simulink library "ammclib_bam_S32K14x"  (R2016a)
settings: Solver=VariableStepAuto  SolverMode=SingleTasking  StartTime=0.0  StopTime=10.0  RelTol=1e-3
undefined symbols (not defined in the file or in its folder): f16A1, f16A2, f16ADCMaxError, f16B0, f16B1, f16B2, f16C1, f16CC1, f16CC1sc, f16CC1sc_D, f16CC1sc_Q, f16CC2, f16CC2sc, f16CC2sc_D, f16CC2sc_Q, f16DerivGain, f16EGain, f16FiltCoef, f16HystOff, f16HystOn, f16IGain, f16IntegGain, f16IntegGainFW, f16IntegGainQ, f16Kd, f16Kq, f16Limit, f16LowerLimit, f16LowerLimit_D, f16LowerLimit_Q, f16LowerLimitFW, f16LowerLimitQ, f16ModIndex, f16OutValOff, f16OutValOn, f16PropGain, f16PropGainFW, f16PropGainQ, f16RampDown, f16RampUp, f16UGain, f16UpperLimit, f16UpperLimit_D, f16UpperLimit_Q, f16UpperLimitFW, f16UpperLimitQ, f16WIGain, f32A1, f32A2, f32ADCMaxError, f32B0, f32B1, f32B2, f32C1, f32CC1, f32CC1sc, f32CC1sc_D, f32CC1sc_Q, f32CC2, f32CC2sc ... (+114)
(part 13 of 22)

== system ammclib_bam_S32K14x/GFLIB/FLT ==
  GFLIB_Acos_FLT : Subsystem  TreatAsAtomicUnit=on  mask(GFLIB_Acos_FLT){}
      mask help: Inverse cosine function in single precision floating-point implementation. Refer to the AMMCLIB User's Guide for further details.
      mask init: same as ammclib_bam_S32K14x/GDFLIB/F16/GDFLIB_FilterFIR_F16
      settings: RTWSystemCode=Inline
      mask Help: web([fileparts(which('ammclib_bam_S32K14x.slx')) '/../doc/S32K14XMCLUG.pdf'], '-browser')
      mask Display: pos = get_param(gcb, 'Position');width = pos(3) - pos(1); height = pos(4) - pos(2);tX=width/2;tY=height - 8;color('black');text(tX,tY, 'GFLIB_Acos_FLT', 'horizontalAlignment', 'center');
  GFLIB_Asin_FLT : Subsystem  TreatAsAtomicUnit=on  mask(GFLIB_Asin_FLT){}
      mask help: Inverse sine function in single precision floating-point implementation. Refer to the AMMCLIB User's Guide for further details.
      mask init: same as ammclib_bam_S32K14x/GDFLIB/F16/GDFLIB_FilterFIR_F16
      settings: RTWSystemCode=Inline
      mask Help: web([fileparts(which('ammclib_bam_S32K14x.slx')) '/../doc/S32K14XMCLUG.pdf'], '-browser')
      mask Display: pos = get_param(gcb, 'Position');width = pos(3) - pos(1); height = pos(4) - pos(2);tX=width/2;tY=height - 8;color('black');text(tX,tY, 'GFLIB_Asin_FLT', 'horizontalAlignment', 'center');
  GFLIB_AtanYXShifted_FLT : Subsystem  TreatAsAtomicUnit=on  mask(GFLIB_AtanYXShifted_FLT){}
      mask help: Shifted arctangent of two arguments Y/X in single precision floating-point implementation. Refer to the AMMCLIB User's Guide for further details.
      mask init: same as ammclib_bam_S32K14x/GDFLIB/F16/GDFLIB_FilterFIR_F16
      settings: RTWSystemCode=Inline
      mask Help: web([fileparts(which('ammclib_bam_S32K14x.slx')) '/../doc/S32K14XMCLUG.pdf'], '-browser')
      mask Display: pos = get_param(gcb, 'Position');width = pos(3) - pos(1); height = pos(4) - pos(2);tX=width/2;tY=height - 8;color('black');text(tX,tY, 'GFLIB_AtanYXShifted_FLT', 'horizontalAlignment', 'center');
  GFLIB_AtanYX_FLT : Subsystem  TreatAsAtomicUnit=on  mask(GFLIB_AtanYX_FLT){}
      mask help: Arctangent of two arguments Y/X in single precision floating-point implementation. Refer to the AMMCLIB User's Guide for further details.
      mask init: same as ammclib_bam_S32K14x/GDFLIB/F16/GDFLIB_FilterFIR_F16
      settings: RTWSystemCode=Inline
      mask Help: web([fileparts(which('ammclib_bam_S32K14x.slx')) '/../doc/S32K14XMCLUG.pdf'], '-browser')
      mask Display: pos = get_param(gcb, 'Position');width = pos(3) - pos(1); height = pos(4) - pos(2);tX=width/2;tY=height - 8;color('black');text(tX,tY, 'GFLIB_AtanYX_FLT', 'horizontalAlignment', 'center');
  GFLIB_Atan_FLT : Subsystem  TreatAsAtomicUnit=on  mask(GFLIB_Atan_FLT){}
      mask help: Inverse tangent function in single precision floating-point implementation. Refer to the AMMCLIB User's Guide for further details.
      mask init: same as ammclib_bam_S32K14x/GDFLIB/F16/GDFLIB_FilterFIR_F16
      settings: RTWSystemCode=Inline
      mask Help: web([fileparts(which('ammclib_bam_S32K14x.slx')) '/../doc/S32K14XMCLUG.pdf'], '-browser')
      mask Display: pos = get_param(gcb, 'Position');width = pos(3) - pos(1); height = pos(4) - pos(2);tX=width/2;tY=height - 8;color('black');text(tX,tY, 'GFLIB_Atan_FLT', 'horizontalAlignment', 'center');
  GFLIB_ControllerPIDpAW_FLT : Subsystem  TreatAsAtomicUnit=on  mask(GFLIB_ControllerPIDpAW_FLT){showStates=Hide (faster execution), resetStatesEnable=Pre-set according to the first set of inputs after reset, fltPropGain=0, fltIntegGain=0, fltDerivGain=0, fltFiltCoef=0, fltLowerLimit=0, fltUpperLimit=0}
      mask prompts: showStates "Show internal states"; resetStatesEnable "Internal state after reset"; fltPropGain "fltPropGain (Proportional gain)"; fltIntegGain "fltIntegGain (Integral gain)"; fltDerivGain "fltDerivGain (Derivative Gain)"; fltFiltCoef "fltFiltCoef (Derivative term filter coefficient)"; fltLowerLimit "fltLowerLimit (Lower Limit of the controller)"; fltUpperLimit "fltUpperLimit (Upper Limit of the controller)"
      mask help: Parallel form PID controller with anti-windup in single precision floating-point implementation. This block supports re-initialization of the internal state during simulation. If the block is reset, the controller's output will be aligned with the input fltControllerPIDpAWOut_preset. Refer to the AMMCLIB User's Guide for further details.
      mask init:
      | if ~evalin('base','exist(''tS8'',''var'')')
      |   if (2 ~= exist('SWLIBS_Typedefs.mat','file'))
      |       error('File SWLIBS_Typedefs.mat is not on the Matlab path. Please add the AMMCLIB "bam" folder in the Matlab Search Path.');
      |   else
      |       evalin('base', 'load(''SWLIBS_Typedefs.mat'')');
      |   end
      | end
      | if showStates == 1
      |     % hidden state variables
      |     if strcmp(get_param([gcb '/fltPropGain'], 'BlockType'), 'Inport')
      |         posblk = get_param(gcb, 'Position');
      | 
      |         pos = get_param(    [gcb, '/fltPropGain'], 'Position');
      |         orient = get_param( [gcb, '/fltPropGain'], 'Orientation');
      |         delete_block(       [gcb, '/fltPropGain']);
      |         add_block('built-in/Ground', [gcb, '/fltPropGain'], 'Position', pos, 'Orientation', orient);
      | 
      |         pos = get_param(    [gcb, '/fltIntegGain'], 'Position');
      |         orient = get_param( [gcb, '/fltIntegGain'], 'Orientation');
      |         delete_block(       [gcb, '/fltIntegGain']);
      |         add_block('built-in/Ground', [gcb, '/fltIntegGain'], 'Position', pos, 'Orientation', orient);
      | 
      |         pos = get_param(    [gcb, '/fltDerivGain'], 'Position');
      |         orient = get_param( [gcb, '/fltDerivGain'], 'Orientation');
      |         delete_block(       [gcb, '/fltDerivGain']);
      |         add_block('built-in/Ground', [gcb, '/fltDerivGain'], 'Position', pos, 'Orientation', orient);
      | 
      |         pos = get_param(    [gcb, '/fltFiltCoef'], 'Position');
      |         orient = get_param( [gcb, '/fltFiltCoef'], 'Orientation');
      |         delete_block(       [gcb, '/fltFiltCoef']);
      |         add_block('built-in/Ground', [gcb, '/fltFiltCoef'], 'Position', pos, 'Orientation', orient);
      | 
      |         pos = get_param(    [gcb, '/fltLowerLimit'], 'Position');
      |         orient = get_param( [gcb, '/fltLowerLimit'], 'Orientation');
      |         delete_block(       [gcb, '/fltLowerLimit']);
      |         add_block('built-in/Ground', [gcb, '/fltLowerLimit'], 'Position', pos, 'Orientation', orient);
      | 
      |         pos = get_param(    [gcb, '/fltUpperLimit'], 'Position');
      |         orient = get_param( [gcb, '/fltUpperLimit'], 'Orientation');
      |         delete_block(       [gcb, '/fltUpperLimit']);
      |         add_block('built-in/Ground', [gcb, '/fltUpperLimit'], 'Position', pos, 'Orientation', orient);
      | 
      |         pos = get_param(    [gcb, '/fltIntegPartK_1'], 'Position');
      |         orient = get_param( [gcb, '/fltIntegPartK_1'], 'Orientation');
      |         delete_block(       [gcb, '/fltIntegPartK_1']);
      |         add_block('built-in/Ground', [gcb, '/fltIntegPartK_1'], 'Position', pos, 'Orientation', orient);
      | 
      |         pos = get_param(    [gcb, '/fltDerivPartK_1'], 'Position');
      |         orient = get_param( [gcb, '/fltDerivPartK_1'], 'Orientation');
      |         delete_block(       [gcb, '/fltDerivPartK_1']);
      |         add_block('built-in/Ground', [gcb, '/fltDerivPartK_1'], 'Position', pos, 'Orientation', orient);
      | 
      |         pos = get_param(    [gcb, '/fltInK_1'], 'Position');
      |         orient = get_param( [gcb, '/fltInK_1'], 'Orientation');
      |         delete_block(       [gcb, '/fltInK_1']);
      |         add_block('built-in/Ground', [gcb, '/fltInK_1'], 'Position', pos, 'Orientation', orient);
      | 
      | 
      |         pos = get_param(    [gcb '/fltIntegPartK_1_Out'], 'Position');
      |         orient = get_param( [gcb '/fltIntegPartK_1_Out'], 'Orientation');
      |         delete_block(       [gcb '/fltIntegPartK_1_Out']);
      |         add_block('built-in/Terminator', [gcb '/fltIntegPartK_1_Out'], 'Position', pos, 'Orientation', orient);
      | 
      |         pos = get_param(    [gcb '/fltDerivPartK_1_Out'], 'Position');
      |         orient = get_param( [gcb '/fltDerivPartK_1_Out'], 'Orientation');
      |         delete_block(       [gcb '/fltDerivPartK_1_Out']);
      |         add_block('built-in/Terminator', [gcb '/fltDerivPartK_1_Out'], 'Position', pos, 'Orientation', orient);
      | 
      |         pos = get_param(    [gcb '/fltInK_1_Out'], 'Position');
      |         orient = get_param( [gcb '/fltInK_1_Out'], 'Orientation');
      |         delete_block(       [gcb '/fltInK_1_Out']);
      |         add_block('built-in/Terminator', [gcb '/fltInK_1_Out'], 'Position', pos, 'Orientation', orient);
      | 
      | 
      |         set_param([gcb '/fltInErr'], 'Port', '1');
      |         set_param([gcb '/fltControllerPIDpAWOut_preset'], 'Port', '2');
      | 
      |         set_param([gcb '/fltOut'], 'Port', '1');
      |         set_param([gcb '/u16LimitFlag'], 'Port', '2');
      | 
      |         set_param(gcb,'MaskEnables',{'on','on','on','on','on','on','on','on'});
      | 
      |         if (posblk(4) - posblk(2)) > 75
      |           height = 75;
      |           set_param(gcb,'Position',[posblk(1), posblk(2), posblk(3), posblk(2)+height])
      |         end
      |     end
      | else
      |     % shown state variables
      |     if strcmp(get_param([gcb '/fltPropGain'], 'BlockType'), 'Ground')
      |         posblk = get_param(gcb, 'Position');
      | 
      |         pos = get_param(    [gcb, '/fltPropGain'], 'Position');
      |         orient = get_param( [gcb, '/fltPropGain'], 'Orientation');
      |         delete_block(       [gcb, '/fltPropGain']);
      |         add_block('built-in/Inport', [gcb, '/fltPropGain'], 'Position', pos, 'Orientation', orient, 'OutDataTypeStr', 'single');
      | 
      |         pos = get_param(    [gcb, '/fltIntegGain'], 'Position');
      |         orient = get_param( [gcb, '/fltIntegGain'], 'Orientation');
      |         delete_block(       [gcb, '/fltIntegGain']);
      |         add_block('built-in/Inport', [gcb, '/fltIntegGain'], 'Position', pos, 'Orientation', orient, 'OutDataTypeStr', 'single');
      | 
      |         pos = get_param(    [gcb, '/fltDerivGain'], 'Position');
      |         orient = get_param( [gcb, '/fltDerivGain'], 'Orientation');
      |         delete_block(       [gcb, '/fltDerivGain']);
      |         add_block('built-in/Inport', [gcb, '/fltDerivGain'], 'Position', pos, 'Orientation', orient, 'OutDataTypeStr', 'single');
      | 
      |         pos = get_param(    [gcb, '/fltFiltCoef'], 'Position');
      |         orient = get_param( [gcb, '/fltFiltCoef'], 'Orientation');
      |         delete_block(       [gcb, '/fltFiltCoef']);
      |         add_block('built-in/Inport', [gcb, '/fltFiltCoef'], 'Position', pos, 'Orientation', orient, 'OutDataTypeStr', 'single');
      | 
      |         pos = get_param(    [gcb, '/fltLowerLimit'], 'Position');
      |         orient = get_param( [gcb, '/fltLowerLimit'], 'Orientation');
      |         delete_block(       [gcb, '/fltLowerLimit']);
      |         add_block('built-in/Inport', [gcb, '/fltLowerLimit'], 'Position', pos, 'Orientation', orient, 'OutDataTypeStr', 'single');
      | 
      |         pos = get_param(    [gcb, '/fltUpperLimit'], 'Position');
      |         orient = get_param( [gcb, '/fltUpperLimit'], 'Orientation');
      |         delete_block(       [gcb, '/fltUpperLimit']);
      |         add_block('built-in/Inport', [gcb, '/fltUpperLimit'], 'Position', pos, 'Orientation', orient, 'OutDataTypeStr', 'single');
      | 
      |         pos = get_param(    [gcb, '/fltIntegPartK_1'], 'Position');
      |         orient = get_param( [gcb, '/fltIntegPartK_1'], 'Orientation');
      |         delete_block(       [gcb, '/fltIntegPartK_1']);
      |         add_block('built-in/Inport', [gcb, '/fltIntegPartK_1'], 'Position', pos, 'Orientation', orient, 'OutDataTypeStr', 'single');
      | 
      |         pos = get_param(    [gcb, '/fltDerivPartK_1'], 'Position');
      |         orient = get_param( [gcb, '/fltDerivPartK_1'], 'Orientation');
      |         delete_block(       [gcb, '/fltDerivPartK_1']);
      |         add_block('built-in/Inport', [gcb, '/fltDerivPartK_1'], 'Position', pos, 'Orientation', orient, 'OutDataTypeStr', 'single');
      | 
      |         pos = get_param(    [gcb, '/fltInK_1'], 'Position');
      |         orient = get_param( [gcb, '/fltInK_1'], 'Orientation');
      |         delete_block(       [gcb, '/fltInK_1']);
      |         add_block('built-in/Inport', [gcb, '/fltInK_1'], 'Position', pos, 'Orientation', orient, 'OutDataTypeStr', 'single');
      | 
      | 
      |         pos = get_param(    [gcb '/fltIntegPartK_1_Out'], 'Position');
      |         orient = get_param( [gcb '/fltIntegPartK_1_Out'], 'Orientation');
      |         delete_block(       [gcb '/fltIntegPartK_1_Out']);
      |         add_block('built-in/Outport', [gcb '/fltIntegPartK_1_Out'], 'Position', pos, 'Orientation', orient);
      | 
      |         pos = get_param(    [gcb '/fltDerivPartK_1_Out'], 'Position');
      |         orient = get_param( [gcb '/fltDerivPartK_1_Out'], 'Orientation');
      |         delete_block(       [gcb '/fltDerivPartK_1_Out']);
      |         add_block('built-in/Outport', [gcb '/fltDerivPartK_1_Out'], 'Position', pos, 'Orientation', orient);
      | 
      |         pos = get_param(    [gcb '/fltInK_1_Out'], 'Position');
      |         orient = get_param( [gcb '/fltInK_1_Out'], 'Orientation');
      |         delete_block(       [gcb '/fltInK_1_Out']);
      |         add_block('built-in/Outport', [gcb '/fltInK_1_Out'], 'Position', pos, 'Orientation', orient);
      | 
      | 
      |         set_param([gcb '/fltInErr'], 'Port', '1');
      |         set_param([gcb '/fltControllerPIDpAWOut_preset'], 'Port', '2');
      |         set_param([gcb '/fltPropGain'], 'Port', '3');
      |         set_param([gcb '/fltIntegGain'], 'Port', '4');
      |         set_param([gcb '/fltDerivGain'], 'Port', '5');
      |         set_param([gcb '/fltFiltCoef'], 'Port', '6');
      |         set_param([gcb '/fltLowerLimit'], 'Port', '7');
      |         set_param([gcb '/fltUpperLimit'], 'Port', '8');
      |         set_param([gcb '/fltIntegPartK_1'], 'Port', '9');
      |         set_param([gcb '/fltDerivPartK_1'], 'Port', '10');
      |         set_param([gcb '/fltInK_1'], 'Port', '11');
      | 
      |         set_param([gcb '/fltOut'], 'Port', '1');
      |         set_param([gcb '/u16LimitFlag'], 'Port', '2');
      |         set_param([gcb '/fltIntegPartK_1_Out'], 'Port', '3');
      |         set_param([gcb '/fltDerivPartK_1_Out'], 'Port', '4');
      |         set_param([gcb '/fltInK_1_Out'], 'Port', '5');
      | 
      |         set_param(gcb,'MaskEnables',{'on','on','off','off','off','off','off','off'});
      | 
      |         if (posblk(4) - posblk(2)) < 300
      |           height = 300;
      |           set_param(gcb,'Position',[posblk(1), posblk(2), posblk(3), posblk(2)+height])
      |         end
      |     end
      | end
      settings: RTWSystemCode=Inline
      mask Help: web([fileparts(which('ammclib_bam_S32K14x.slx')) '/../doc/S32K14XMCLUG.pdf'], '-browser')
      mask TypeOptions showStates: Hide (faster execution) | Show (allows debugging; connect feedback loops manually)
      mask Callback showStates:
      | maskStr = get_param(gcb,'showStates');
      | if strcmp(maskStr,'Hide (faster execution)'),
      |     set_param(gcb,'MaskEnables',{'on','on','on','on','on','on','on','on'});
      | else
      |     set_param(gcb,'MaskEnables',{'on','on','off','off','off','off','off','off'});
      | end
      mask TypeOptions resetStatesEnable: Pre-set according to the first set of inputs after reset | Clear to zero
      mask Display:
      | color('black');
      | pos = get_param(gcb, 'Position');
      | width = pos(3) - pos(1);
      | height = pos(4) - pos(2);
      | tX=width/2;
      | tY=height - 25;
      | color('black');
      | text(tX,tY, 'GFLIB_ControllerPIDpAW_FLT', 'horizontalAlignment', 'center');
      | if showStates == 2
      |   color('red');
      |   text(tX,tY - 20, ['debugging mode' char(13) char(10) '(limited performance)'], 'horizontalAlignment', 'center');
      | end
  GFLIB_ControllerPIpAW_FLT : Subsystem  TreatAsAtomicUnit=on  mask(GFLIB_ControllerPIpAW_FLT){showStates=Hide (faster execution), resetStatesEnable=Pre-set according to the first set of inputs after reset, fltPropGain=0, fltIntegGain=0, fltLowerLimit=0, fltUpperLimit=0}
      mask prompts: showStates "Show internal states"; resetStatesEnable "Internal state after reset"; fltPropGain "fltPropGain (Proportional gain)"; fltIntegGain "fltIntegGain (Integral gain)"; fltLowerLimit "fltLowerLimit (Lower Limit of the controller)"; fltUpperLimit "fltUpperLimit (Upper Limit of the controller)"
      mask help: Parallel form PI controller with anti-windup in single precision floating-point implementation. This block supports re-initialization of the internal state during simulation. If the block is reset, the controller's output will be aligned with the input fltControllerPIpAWOut_preset. Refer to the AMMCLIB User's Guide for further details.
      mask init:
      | if ~evalin('base','exist(''tS8'',''var'')')
      |   if (2 ~= exist('SWLIBS_Typedefs.mat','file'))
      |       error('File SWLIBS_Typedefs.mat is not on the Matlab path. Please add the AMMCLIB "bam" folder in the Matlab Search Path.');
      |   else
      |       evalin('base', 'load(''SWLIBS_Typedefs.mat'')');
      |   end
      | end
      | if showStates == 1
      |     % hidden state variables
      |     if strcmp(get_param([gcb '/fltPropGain'], 'BlockType'), 'Inport')
      |         posblk = get_param(gcb, 'Position');
      | 
      |         pos = get_param(    [gcb, '/fltPropGain'], 'Position');
      |         orient = get_param( [gcb, '/fltPropGain'], 'Orientation');
      |         delete_block(       [gcb, '/fltPropGain']);
      |         add_block('built-in/Ground', [gcb, '/fltPropGain'], 'Position', pos, 'Orientation', orient);
      | 
      |         pos = get_param(    [gcb, '/fltIntegGain'], 'Position');
      |         orient = get_param( [gcb, '/fltIntegGain'], 'Orientation');
      |         delete_block(       [gcb, '/fltIntegGain']);
      |         add_block('built-in/Ground', [gcb, '/fltIntegGain'], 'Position', pos, 'Orientation', orient);
      | 
      |         pos = get_param(    [gcb, '/fltLowerLimit'], 'Position');
      |         orient = get_param( [gcb, '/fltLowerLimit'], 'Orientation');
      |         delete_block(       [gcb, '/fltLowerLimit']);
      |         add_block('built-in/Ground', [gcb, '/fltLowerLimit'], 'Position', pos, 'Orientation', orient);
      | 
      |         pos = get_param(    [gcb, '/fltUpperLimit'], 'Position');
      |         orient = get_param( [gcb, '/fltUpperLimit'], 'Orientation');
      |         delete_block(       [gcb, '/fltUpperLimit']);
      |         add_block('built-in/Ground', [gcb, '/fltUpperLimit'], 'Position', pos, 'Orientation', orient);
      | 
      |         pos = get_param(    [gcb, '/fltIntegPartK_1'], 'Position');
      |         orient = get_param( [gcb, '/fltIntegPartK_1'], 'Orientation');
      |         delete_block(       [gcb, '/fltIntegPartK_1']);
      |         add_block('built-in/Ground', [gcb, '/fltIntegPartK_1'], 'Position', pos, 'Orientation', orient);
      | 
      |         pos = get_param(    [gcb, '/fltInK_1'], 'Position');
      |         orient = get_param( [gcb, '/fltInK_1'], 'Orientation');
      |         delete_block(       [gcb, '/fltInK_1']);
      |         add_block('built-in/Ground', [gcb, '/fltInK_1'], 'Position', pos, 'Orientation', orient);
      | 
      | 
      |         pos = get_param(    [gcb '/fltIntegPartK_1_Out'], 'Position');
      |         orient = get_param( [gcb '/fltIntegPartK_1_Out'], 'Orientation');
      |         delete_block(       [gcb '/fltIntegPartK_1_Out']);
      |         add_block('built-in/Terminator', [gcb '/fltIntegPartK_1_Out'], 'Position', pos, 'Orientation', orient);
      | 
      |         pos = get_param(    [gcb '/fltInK_1_Out'], 'Position');
      |         orient = get_param( [gcb '/fltInK_1_Out'], 'Orientation');
      |         delete_block(       [gcb '/fltInK_1_Out']);
      |         add_block('built-in/Terminator', [gcb '/fltInK_1_Out'], 'Position', pos, 'Orientation', orient);
      | 
      | 
      |         set_param([gcb '/fltInErr'], 'Port', '1');
      |         set_param([gcb '/fltControllerPIpAWOut_preset'], 'Port', '2');
      | 
      |         set_param([gcb '/fltOut'], 'Port', '1');
      |         set_param([gcb '/u16LimitFlag'], 'Port', '2');
      | 
      |         set_param(gcb,'MaskEnables',{'on','on','on','on','on','on'});
      | 
      |         if (posblk(4) - posblk(2)) > 75
      |           height = 75;
      |           set_param(gcb,'Position',[posblk(1), posblk(2), posblk(3), posblk(2)+height])
      |         end
      |     end
      | else
      |     % shown state variables
      |     if strcmp(get_param([gcb '/fltPropGain'], 'BlockType'), 'Ground')
      |         posblk = get_param(gcb, 'Position');
      | 
      |         pos = get_param(    [gcb, '/fltPropGain'], 'Position');
      |         orient = get_param( [gcb, '/fltPropGain'], 'Orientation');
      |         delete_block(       [gcb, '/fltPropGain']);
      |         add_block('built-in/Inport', [gcb, '/fltPropGain'], 'Position', pos, 'Orientation', orient, 'OutDataTypeStr', 'single');
      | 
      |         pos = get_param(    [gcb, '/fltIntegGain'], 'Position');
      |         orient = get_param( [gcb, '/fltIntegGain'], 'Orientation');
      |         delete_block(       [gcb, '/fltIntegGain']);
      |         add_block('built-in/Inport', [gcb, '/fltIntegGain'], 'Position', pos, 'Orientation', orient, 'OutDataTypeStr', 'single');
      | 
      |         pos = get_param(    [gcb, '/fltLowerLimit'], 'Position');
      |         orient = get_param( [gcb, '/fltLowerLimit'], 'Orientation');
      |         delete_block(       [gcb, '/fltLowerLimit']);
      |         add_block('built-in/Inport', [gcb, '/fltLowerLimit'], 'Position', pos, 'Orientation', orient, 'OutDataTypeStr', 'single');
      | 
      |         pos = get_param(    [gcb, '/fltUpperLimit'], 'Position');
      |         orient = get_param( [gcb, '/fltUpperLimit'], 'Orientation');
      |         delete_block(       [gcb, '/fltUpperLimit']);
      |         add_block('built-in/Inport', [gcb, '/fltUpperLimit'], 'Position', pos, 'Orientation', orient, 'OutDataTypeStr', 'single');
      | 
      |         pos = get_param(    [gcb, '/fltIntegPartK_1'], 'Position');
      |         orient = get_param( [gcb, '/fltIntegPartK_1'], 'Orientation');
      |         delete_block(       [gcb, '/fltIntegPartK_1']);
      |         add_block('built-in/Inport', [gcb, '/fltIntegPartK_1'], 'Position', pos, 'Orientation', orient, 'OutDataTypeStr', 'single');
      | 
      |         pos = get_param(    [gcb, '/fltInK_1'], 'Position');
      |         orient = get_param( [gcb, '/fltInK_1'], 'Orientation');
      |         delete_block(       [gcb, '/fltInK_1']);
      |         add_block('built-in/Inport', [gcb, '/fltInK_1'], 'Position', pos, 'Orientation', orient, 'OutDataTypeStr', 'single');
      | 
      | 
      |         pos = get_param(    [gcb '/fltIntegPartK_1_Out'], 'Position');
      |         orient = get_param( [gcb '/fltIntegPartK_1_Out'], 'Orientation');
      |         delete_block(       [gcb '/fltIntegPartK_1_Out']);
      |         add_block('built-in/Outport', [gcb '/fltIntegPartK_1_Out'], 'Position', pos, 'Orientation', orient);
      | 
      |         pos = get_param(    [gcb '/fltInK_1_Out'], 'Position');
      |         orient = get_param( [gcb '/fltInK_1_Out'], 'Orientation');
      |         delete_block(       [gcb '/fltInK_1_Out']);
      |         add_block('built-in/Outport', [gcb '/fltInK_1_Out'], 'Position', pos, 'Orientation', orient);
      | 
      | 
      |         set_param([gcb '/fltInErr'], 'Port', '1');
      |         set_param([gcb '/fltControllerPIpAWOut_preset'], 'Port', '2');
      |         set_param([gcb '/fltPropGain'], 'Port', '3');
      |         set_param([gcb '/fltIntegGain'], 'Port', '4');
      |         set_param([gcb '/fltLowerLimit'], 'Port', '5');
      |         set_param([gcb '/fltUpperLimit'], 'Port', '6');
      |         set_param([gcb '/fltIntegPartK_1'], 'Port', '7');
      |         set_param([gcb '/fltInK_1'], 'Port', '8');
      | 
      |         set_param([gcb '/fltOut'], 'Port', '1');
      |         set_param([gcb '/u16LimitFlag'], 'Port', '2');
      |         set_param([gcb '/fltIntegPartK_1_Out'], 'Port', '3');
      |         set_param([gcb '/fltInK_1_Out'], 'Port', '4');
      | 
      |         set_param(gcb,'MaskEnables',{'on','on','off','off','off','off'});
      | 
      |         if (posblk(4) - posblk(2)) < 225
      |           height = 225;
      |           set_param(gcb,'Position',[posblk(1), posblk(2), posblk(3), posblk(2)+height])
      |         end
      |     end
      | end
      settings: RTWSystemCode=Inline
      mask Help: web([fileparts(which('ammclib_bam_S32K14x.slx')) '/../doc/S32K14XMCLUG.pdf'], '-browser')
      mask TypeOptions showStates: Hide (faster execution) | Show (allows debugging; connect feedback loops manually)
      mask Callback showStates:
      | maskStr = get_param(gcb,'showStates');
      | if strcmp(maskStr,'Hide (faster execution)'),
      |     set_param(gcb,'MaskEnables',{'on','on','on','on','on','on'});
      | else
      |     set_param(gcb,'MaskEnables',{'on','on','off','off','off','off'});
      | end
      mask TypeOptions resetStatesEnable: Pre-set according to the first set of inputs after reset | Clear to zero
      mask Display:
      | color('black');
      | pos = get_param(gcb, 'Position');
      | width = pos(3) - pos(1);
      | height = pos(4) - pos(2);
      | tX=width/2;
      | tY=height - 25;
      | color('black');
      | text(tX,tY, 'GFLIB_ControllerPIpAW_FLT', 'horizontalAlignment', 'center');
      | if showStates == 2
      |   color('red');
      |   text(tX,tY - 20, ['debugging mode' char(13) char(10) '(limited performance)'], 'horizontalAlignment', 'center');
      | end
  GFLIB_ControllerPIp_FLT : Subsystem  TreatAsAtomicUnit=on  mask(GFLIB_ControllerPIp_FLT){showStates=Hide (faster execution), resetStatesEnable=Pre-set according to the first set of inputs after reset, fltPropGain=0, fltIntegGain=0}
      mask prompts: showStates "Show internal states"; resetStatesEnable "Internal state after reset"; fltPropGain "fltPropGain (Proportional gain)"; fltIntegGain "fltIntegGain (Integral gain)"
      mask help: Parallel form PI controller without anti-windup in single precision floating-point implementation. This block supports re-initialization of the internal state during simulation. If the block is reset, the controller's output will be aligned with the input fltControllerPIpOut_preset. Refer to the AMMCLIB User's Guide for further details.
      mask init:
      | if ~evalin('base','exist(''tS8'',''var'')')
      |   if (2 ~= exist('SWLIBS_Typedefs.mat','file'))
      |       error('File SWLIBS_Typedefs.mat is not on the Matlab path. Please add the AMMCLIB "bam" folder in the Matlab Search Path.');
      |   else
      |       evalin('base', 'load(''SWLIBS_Typedefs.mat'')');
      |   end
      | end
      | if showStates == 1
      |     % hidden state variables
      |     if strcmp(get_param([gcb '/fltPropGain'], 'BlockType'), 'Inport')
      |         posblk = get_param(gcb, 'Position');
      | 
      |         pos = get_param(    [gcb, '/fltPropGain'], 'Position');
      |         orient = get_param( [gcb, '/fltPropGain'], 'Orientation');
      |         delete_block(       [gcb, '/fltPropGain']);
      |         add_block('built-in/Ground', [gcb, '/fltPropGain'], 'Position', pos, 'Orientation', orient);
      | 
      |         pos = get_param(    [gcb, '/fltIntegGain'], 'Position');
      |         orient = get_param( [gcb, '/fltIntegGain'], 'Orientation');
      |         delete_block(       [gcb, '/fltIntegGain']);
      |         add_block('built-in/Ground', [gcb, '/fltIntegGain'], 'Position', pos, 'Orientation', orient);
      | 
      |         pos = get_param(    [gcb, '/fltIntegPartK_1'], 'Position');
      |         orient = get_param( [gcb, '/fltIntegPartK_1'], 'Orientation');
      |         delete_block(       [gcb, '/fltIntegPartK_1']);
      |         add_block('built-in/Ground', [gcb, '/fltIntegPartK_1'], 'Position', pos, 'Orientation', orient);
      | 
      |         pos = get_param(    [gcb, '/fltInK_1'], 'Position');
      |         orient = get_param( [gcb, '/fltInK_1'], 'Orientation');
      |         delete_block(       [gcb, '/fltInK_1']);
      |         add_block('built-in/Ground', [gcb, '/fltInK_1'], 'Position', pos, 'Orientation', orient);
      | 
      | 
      |         pos = get_param(    [gcb '/fltIntegPartK_1_Out'], 'Position');
      |         orient = get_param( [gcb '/fltIntegPartK_1_Out'], 'Orientation');
      |         delete_block(       [gcb '/fltIntegPartK_1_Out']);
      |         add_block('built-in/Terminator', [gcb '/fltIntegPartK_1_Out'], 'Position', pos, 'Orientation', orient);
      | 
      |         pos = get_param(    [gcb '/fltInK_1_Out'], 'Position');
      |         orient = get_param( [gcb '/fltInK_1_Out'], 'Orientation');
      |         delete_block(       [gcb '/fltInK_1_Out']);
      |         add_block('built-in/Terminator', [gcb '/fltInK_1_Out'], 'Position', pos, 'Orientation', orient);
      | 
      | 
      |         set_param([gcb '/fltInErr'], 'Port', '1');
      |         set_param([gcb '/fltControllerPIpOut_preset'], 'Port', '2');
      | 
      |         set_param([gcb '/fltOut'], 'Port', '1');
      | 
      |         set_param(gcb,'MaskEnables',{'on','on','on','on'});
      | 
      |         if (posblk(4) - posblk(2)) > 75
      |           height = 75;
      |           set_param(gcb,'Position',[posblk(1), posblk(2), posblk(3), posblk(2)+height])
      |         end
      |     end
      | else
      |     % shown state variables
      |     if strcmp(get_param([gcb '/fltPropGain'], 'BlockType'), 'Ground')
      |         posblk = get_param(gcb, 'Position');
      | 
      |         pos = get_param(    [gcb, '/fltPropGain'], 'Position');
      |         orient = get_param( [gcb, '/fltPropGain'], 'Orientation');
      |         delete_block(       [gcb, '/fltPropGain']);
      |         add_block('built-in/Inport', [gcb, '/fltPropGain'], 'Position', pos, 'Orientation', orient, 'OutDataTypeStr', 'single');
      | 
      |         pos = get_param(    [gcb, '/fltIntegGain'], 'Position');
      |         orient = get_param( [gcb, '/fltIntegGain'], 'Orientation');
      |         delete_block(       [gcb, '/fltIntegGain']);
      |         add_block('built-in/Inport', [gcb, '/fltIntegGain'], 'Position', pos, 'Orientation', orient, 'OutDataTypeStr', 'single');
      | 
      |         pos = get_param(    [gcb, '/fltIntegPartK_1'], 'Position');
      |         orient = get_param( [gcb, '/fltIntegPartK_1'], 'Orientation');
      |         delete_block(       [gcb, '/fltIntegPartK_1']);
      |         add_block('built-in/Inport', [gcb, '/fltIntegPartK_1'], 'Position', pos, 'Orientation', orient, 'OutDataTypeStr', 'single');
      | 
      |         pos = get_param(    [gcb, '/fltInK_1'], 'Position');
      |         orient = get_param( [gcb, '/fltInK_1'], 'Orientation');
      |         delete_block(       [gcb, '/fltInK_1']);
      |         add_block('built-in/Inport', [gcb, '/fltInK_1'], 'Position', pos, 'Orientation', orient, 'OutDataTypeStr', 'single');
      | 
      | 
      |         pos = get_param(    [gcb '/fltIntegPartK_1_Out'], 'Position');
      |         orient = get_param( [gcb '/fltIntegPartK_1_Out'], 'Orientation');
      |         delete_block(       [gcb '/fltIntegPartK_1_Out']);
      |         add_block('built-in/Outport', [gcb '/fltIntegPartK_1_Out'], 'Position', pos, 'Orientation', orient);
      | 
      |         pos = get_param(    [gcb '/fltInK_1_Out'], 'Position');
      |         orient = get_param( [gcb '/fltInK_1_Out'], 'Orientation');
      |         delete_block(       [gcb '/fltInK_1_Out']);
      |         add_block('built-in/Outport', [gcb '/fltInK_1_Out'], 'Position', pos, 'Orientation', orient);
      | 
      | 
      |         set_param([gcb '/fltInErr'], 'Port', '1');
      |         set_param([gcb '/fltControllerPIpOut_preset'], 'Port', '2');
      |         set_param([gcb '/fltPropGain'], 'Port', '3');
      |         set_param([gcb '/fltIntegGain'], 'Port', '4');
      |         set_param([gcb '/fltIntegPartK_1'], 'Port', '5');
      |         set_param([gcb '/fltInK_1'], 'Port', '6');
      | 
      |         set_param([gcb '/fltOut'], 'Port', '1');
      |         set_param([gcb '/fltIntegPartK_1_Out'], 'Port', '2');
      |         set_param([gcb '/fltInK_1_Out'], 'Port', '3');
      | 
      |         set_param(gcb,'MaskEnables',{'on','on','off','off'});
      | 
      |         if (posblk(4) - posblk(2)) < 175
      |           height = 175;
      |           set_param(gcb,'Position',[posblk(1), posblk(2), posblk(3), posblk(2)+height])
      |         end
      |     end
      | end
      settings: RTWSystemCode=Inline
      mask Help: web([fileparts(which('ammclib_bam_S32K14x.slx')) '/../doc/S32K14XMCLUG.pdf'], '-browser')
      mask TypeOptions showStates: Hide (faster execution) | Show (allows debugging; connect feedback loops manually)
      mask Callback showStates:
      | maskStr = get_param(gcb,'showStates');
      | if strcmp(maskStr,'Hide (faster execution)'),
      |     set_param(gcb,'MaskEnables',{'on','on','on','on'});
      | else
      |     set_param(gcb,'MaskEnables',{'on','on','off','off'});
      | end
      mask TypeOptions resetStatesEnable: Pre-set according to the first set of inputs after reset | Clear to zero
      mask Display:
      | color('black');
      | pos = get_param(gcb, 'Position');
      | width = pos(3) - pos(1);
      | height = pos(4) - pos(2);
      | tX=width/2;
      | tY=height - 25;
      | color('black');
      | text(tX,tY, 'GFLIB_ControllerPIp_FLT', 'horizontalAlignment', 'center');
      | if showStates == 2
      |   color('red');
      |   text(tX,tY - 20, ['debugging mode' char(13) char(10) '(limited performance)'], 'horizontalAlignment', 'center');
      | end
  GFLIB_ControllerPIrAW_FLT : Subsystem  TreatAsAtomicUnit=on  mask(GFLIB_ControllerPIrAW_FLT){showStates=Hide (faster execution), resetStatesEnable=Pre-set according to the first set of inputs after reset, fltUpperLimit=0, fltLowerLimit=0, fltCC1sc=0, fltCC2sc=0}
      mask prompts: showStates "Show internal states"; resetStatesEnable "Internal state after reset"; fltUpperLimit "fltUpperLimit (Upper Limit of the controller)"; fltLowerLimit "fltLowerLimit (Lower Limit of the controller)"; fltCC1sc "fltCC1sc (CC1 coefficient)"; fltCC2sc "fltCC2sc (CC2 coefficient)"
      mask help: Recurrent form PI controller with anti-windup in single precision floating-point implementation. This block supports re-initialization of the internal state during simulation. If the block is reset, the controller's output will be aligned with the input fltControllerPIrAWOut_preset. Refer to the AMMCLIB User's Guide for further details.
      mask init:
      | if ~evalin('base','exist(''tS8'',''var'')')
      |   if (2 ~= exist('SWLIBS_Typedefs.mat','file'))
      |       error('File SWLIBS_Typedefs.mat is not on the Matlab path. Please add the AMMCLIB "bam" folder in the Matlab Search Path.');
      |   else
      |       evalin('base', 'load(''SWLIBS_Typedefs.mat'')');
      |   end
      | end
      | if showStates == 1
      |     % hidden state variables
      |     if strcmp(get_param([gcb '/fltUpperLimit'], 'BlockType'), 'Inport')
      |         posblk = get_param(gcb, 'Position');
      | 
      |         pos = get_param(    [gcb, '/fltUpperLimit'], 'Position');
      |         orient = get_param( [gcb, '/fltUpperLimit'], 'Orientation');
      |         delete_block(       [gcb, '/fltUpperLimit']);
      |         add_block('built-in/Ground', [gcb, '/fltUpperLimit'], 'Position', pos, 'Orientation', orient);
      | 
      |         pos = get_param(    [gcb, '/fltLowerLimit'], 'Position');
      |         orient = get_param( [gcb, '/fltLowerLimit'], 'Orientation');
      |         delete_block(       [gcb, '/fltLowerLimit']);
      |         add_block('built-in/Ground', [gcb, '/fltLowerLimit'], 'Position', pos, 'Orientation', orient);
      | 
      |         pos = get_param(    [gcb, '/fltAcc'], 'Position');
      |         orient = get_param( [gcb, '/fltAcc'], 'Orientation');
      |         delete_block(       [gcb, '/fltAcc']);
      |         add_block('built-in/Ground', [gcb, '/fltAcc'], 'Position', pos, 'Orientation', orient);
      | 
      |         pos = get_param(    [gcb, '/fltInErrK1'], 'Position');
      |         orient = get_param( [gcb, '/fltInErrK1'], 'Orientation');
      |         delete_block(       [gcb, '/fltInErrK1']);
      |         add_block('built-in/Ground', [gcb, '/fltInErrK1'], 'Position', pos, 'Orientation', orient);
      | 
      |         pos = get_param(    [gcb, '/fltCC1sc'], 'Position');
      |         orient = get_param( [gcb, '/fltCC1sc'], 'Orientation');
      |         delete_block(       [gcb, '/fltCC1sc']);
      |         add_block('built-in/Ground', [gcb, '/fltCC1sc'], 'Position', pos, 'Orientation', orient);
      | 
      |         pos = get_param(    [gcb, '/fltCC2sc'], 'Position');
      |         orient = get_param( [gcb, '/fltCC2sc'], 'Orientation');
      |         delete_block(       [gcb, '/fltCC2sc']);
      |         add_block('built-in/Ground', [gcb, '/fltCC2sc'], 'Position', pos, 'Orientation', orient);
      | 
      | 
      |         pos = get_param(    [gcb '/fltAcc_Out'], 'Position');
      |         orient = get_param( [gcb '/fltAcc_Out'], 'Orientation');
      |         delete_block(       [gcb '/fltAcc_Out']);
      |         add_block('built-in/Terminator', [gcb '/fltAcc_Out'], 'Position', pos, 'Orientation', orient);
      | 
      |         pos = get_param(    [gcb '/fltInErrK1_Out'], 'Position');
      |         orient = get_param( [gcb '/fltInErrK1_Out'], 'Orientation');
      |         delete_block(       [gcb '/fltInErrK1_Out']);
      |         add_block('built-in/Terminator', [gcb '/fltInErrK1_Out'], 'Position', pos, 'Orientation', orient);
      | 
      | 
      |         set_param([gcb '/fltInErr'], 'Port', '1');
      |         set_param([gcb '/fltControllerPIrAWOut_preset'], 'Port', '2');
      | 
      |         set_param([gcb '/fltOut'], 'Port', '1');
      | 
      |         set_param(gcb,'MaskEnables',{'on','on','on','on','on','on'});
      | 
      |         if (posblk(4) - posblk(2)) > 75
      |           height = 75;
      |           set_param(gcb,'Position',[posblk(1), posblk(2), posblk(3), posblk(2)+height])
      |         end
      |     end
      | else
      |     % shown state variables
      |     if strcmp(get_param([gcb '/fltUpperLimit'], 'BlockType'), 'Ground')
      |         posblk = get_param(gcb, 'Position');
      | 
      |         pos = get_param(    [gcb, '/fltUpperLimit'], 'Position');
      |         orient = get_param( [gcb, '/fltUpperLimit'], 'Orientation');
      |         delete_block(       [gcb, '/fltUpperLimit']);
      |         add_block('built-in/Inport', [gcb, '/fltUpperLimit'], 'Position', pos, 'Orientation', orient, 'OutDataTypeStr', 'single');
      | 
      |         pos = get_param(    [gcb, '/fltLowerLimit'], 'Position');
      |         orient = get_param( [gcb, '/fltLowerLimit'], 'Orientation');
      |         delete_block(       [gcb, '/fltLowerLimit']);
      |         add_block('built-in/Inport', [gcb, '/fltLowerLimit'], 'Position', pos, 'Orientation', orient, 'OutDataTypeStr', 'single');
      | 
      |         pos = get_param(    [gcb, '/fltAcc'], 'Position');
      |         orient = get_param( [gcb, '/fltAcc'], 'Orientation');
      |         delete_block(       [gcb, '/fltAcc']);
      |         add_block('built-in/Inport', [gcb, '/fltAcc'], 'Position', pos, 'Orientation', orient, 'OutDataTypeStr', 'single');
      | 
      |         pos = get_param(    [gcb, '/fltInErrK1'], 'Position');
      |         orient = get_param( [gcb, '/fltInErrK1'], 'Orientation');
      |         delete_block(       [gcb, '/fltInErrK1']);
      |         add_block('built-in/Inport', [gcb, '/fltInErrK1'], 'Position', pos, 'Orientation', orient, 'OutDataTypeStr', 'single');
      | 
      |         pos = get_param(    [gcb, '/fltCC1sc'], 'Position');
      |         orient = get_param( [gcb, '/fltCC1sc'], 'Orientation');
      |         delete_block(       [gcb, '/fltCC1sc']);
      |         add_block('built-in/Inport', [gcb, '/fltCC1sc'], 'Position', pos, 'Orientation', orient, 'OutDataTypeStr', 'single');
      | 
      |         pos = get_param(    [gcb, '/fltCC2sc'], 'Position');
      |         orient = get_param( [gcb, '/fltCC2sc'], 'Orientation');
      |         delete_block(       [gcb, '/fltCC2sc']);
      |         add_block('built-in/Inport', [gcb, '/fltCC2sc'], 'Position', pos, 'Orientation', orient, 'OutDataTypeStr', 'single');
      | 
      | 
      |         pos = get_param(    [gcb '/fltAcc_Out'], 'Position');
      |         orient = get_param( [gcb '/fltAcc_Out'], 'Orientation');
      |         delete_block(       [gcb '/fltAcc_Out']);
      |         add_block('built-in/Outport', [gcb '/fltAcc_Out'], 'Position', pos, 'Orientation', orient);
      | 
      |         pos = get_param(    [gcb '/fltInErrK1_Out'], 'Position');
      |         orient = get_param( [gcb '/fltInErrK1_Out'], 'Orientation');
      |         delete_block(       [gcb '/fltInErrK1_Out']);
      |         add_block('built-in/Outport', [gcb '/fltInErrK1_Out'], 'Position', pos, 'Orientation', orient);
      | 
      | 
      |         set_param([gcb '/fltInErr'], 'Port', '1');
      |         set_param([gcb '/fltControllerPIrAWOut_preset'], 'Port', '2');
      |         set_param([gcb '/fltUpperLimit'], 'Port', '3');
      |         set_param([gcb '/fltLowerLimit'], 'Port', '4');
      |         set_param([gcb '/fltAcc'], 'Port', '5');
      |         set_param([gcb '/fltInErrK1'], 'Port', '6');
      |         set_param([gcb '/fltCC1sc'], 'Port', '7');
      |         set_param([gcb '/fltCC2sc'], 'Port', '8');
      | 
      |         set_param([gcb '/fltOut'], 'Port', '1');
      |         set_param([gcb '/fltAcc_Out'], 'Port', '2');
      |         set_param([gcb '/fltInErrK1_Out'], 'Port', '3');
      | 
      |         set_param(gcb,'MaskEnables',{'on','on','off','off','off','off'});
      | 
      |         if (posblk(4) - posblk(2)) < 225
      |           height = 225;
      |           set_param(gcb,'Position',[posblk(1), posblk(2), posblk(3), posblk(2)+height])
      |         end
      |     end
      | end
      settings: RTWSystemCode=Inline
      mask Help: web([fileparts(which('ammclib_bam_S32K14x.slx')) '/../doc/S32K14XMCLUG.pdf'], '-browser')
      mask TypeOptions showStates: Hide (faster execution) | Show (allows debugging; connect feedback loops manually)
      mask Callback showStates:
      | maskStr = get_param(gcb,'showStates');
      | if strcmp(maskStr,'Hide (faster execution)'),
      |     set_param(gcb,'MaskEnables',{'on','on','on','on','on','on'});
      | else
      |     set_param(gcb,'MaskEnables',{'on','on','off','off','off','off'});
      | end
      mask TypeOptions resetStatesEnable: Pre-set according to the first set of inputs after reset | Clear to zero
      mask Display:
      | color('black');
      | pos = get_param(gcb, 'Position');
      | width = pos(3) - pos(1);
      | height = pos(4) - pos(2);
      | tX=width/2;
      | tY=height - 25;
      | color('black');
      | text(tX,tY, 'GFLIB_ControllerPIrAW_FLT', 'horizontalAlignment', 'center');
      | if showStates == 2
      |   color('red');
      |   text(tX,tY - 20, ['debugging mode' char(13) char(10) '(limited performance)'], 'horizontalAlignment', 'center');
      | end
  GFLIB_ControllerPIr_FLT : Subsystem  TreatAsAtomicUnit=on  mask(GFLIB_ControllerPIr_FLT){showStates=Hide (faster execution), resetStatesEnable=Pre-set according to the first set of inputs after reset, fltCC1=0, fltCC2=0}
      mask prompts: showStates "Show internal states"; resetStatesEnable "Internal state after reset"; fltCC1 "fltCC1 (CC1 coefficient)"; fltCC2 "fltCC2 (CC2 coefficient)"
      mask help: Reccurent form PI controller without anti-windup in single precision floating-point implementation. This block supports re-initialization of the internal state during simulation. If the block is reset, the controller's output will be aligned with the input fltControllerPIrOut_preset. Refer to the AMMCLIB User's Guide for further details.
      mask init:
      | if ~evalin('base','exist(''tS8'',''var'')')
      |   if (2 ~= exist('SWLIBS_Typedefs.mat','file'))
      |       error('File SWLIBS_Typedefs.mat is not on the Matlab path. Please add the AMMCLIB "bam" folder in the Matlab Search Path.');
      |   else
      |       evalin('base', 'load(''SWLIBS_Typedefs.mat'')');
      |   end
      | end
      | if showStates == 1
      |     % hidden state variables
      |     if strcmp(get_param([gcb '/fltCC1sc'], 'BlockType'), 'Inport')
      |         posblk = get_param(gcb, 'Position');
      | 
      |         pos = get_param(    [gcb, '/fltCC1sc'], 'Position');
      |         orient = get_param( [gcb, '/fltCC1sc'], 'Orientation');
      |         delete_block(       [gcb, '/fltCC1sc']);
      |         add_block('built-in/Ground', [gcb, '/fltCC1sc'], 'Position', pos, 'Orientation', orient);
      | 
      |         pos = get_param(    [gcb, '/fltCC2sc'], 'Position');
      |         orient = get_param( [gcb, '/fltCC2sc'], 'Orientation');
      |         delete_block(       [gcb, '/fltCC2sc']);
      |         add_block('built-in/Ground', [gcb, '/fltCC2sc'], 'Position', pos, 'Orientation', orient);
      | 
      |         pos = get_param(    [gcb, '/fltAcc'], 'Position');
      |         orient = get_param( [gcb, '/fltAcc'], 'Orientation');
      |         delete_block(       [gcb, '/fltAcc']);
      |         add_block('built-in/Ground', [gcb, '/fltAcc'], 'Position', pos, 'Orientation', orient);
      | 
      |         pos = get_param(    [gcb, '/fltInErrK1'], 'Position');
      |         orient = get_param( [gcb, '/fltInErrK1'], 'Orientation');
      |         delete_block(       [gcb, '/fltInErrK1']);
      |         add_block('built-in/Ground', [gcb, '/fltInErrK1'], 'Position', pos, 'Orientation', orient);
      | 
      | 
      |         pos = get_param(    [gcb '/fltAcc_Out'], 'Position');
      |         orient = get_param( [gcb '/fltAcc_Out'], 'Orientation');
      |         delete_block(       [gcb '/fltAcc_Out']);
      |         add_block('built-in/Terminator', [gcb '/fltAcc_Out'], 'Position', pos, 'Orientation', orient);
      | 
      |         pos = get_param(    [gcb '/fltInErrK1_Out'], 'Position');
      |         orient = get_param( [gcb '/fltInErrK1_Out'], 'Orientation');
      |         delete_block(       [gcb '/fltInErrK1_Out']);
      |         add_block('built-in/Terminator', [gcb '/fltInErrK1_Out'], 'Position', pos, 'Orientation', orient);
      | 
      | 
      |         set_param([gcb '/fltInErr'], 'Port', '1');
      |         set_param([gcb '/fltControllerPIrOut_preset'], 'Port', '2');
      | 
      |         set_param([gcb '/fltOut'], 'Port', '1');
      | 
      |         set_param(gcb,'MaskEnables',{'on','on','on','on'});
      | 
      |         if (posblk(4) - posblk(2)) > 75
      |           height = 75;
      |           set_param(gcb,'Position',[posblk(1), posblk(2), posblk(3), posblk(2)+height])
      |         end
      |     end
      | else
      |     % shown state variables
      |     if strcmp(get_param([gcb '/fltCC1sc'], 'BlockType'), 'Ground')
      |         posblk = get_param(gcb, 'Position');
      | 
      |         pos = get_param(    [gcb, '/fltCC1sc'], 'Position');
      |         orient = get_param( [gcb, '/fltCC1sc'], 'Orientation');
      |         delete_block(       [gcb, '/fltCC1sc']);
      |         add_block('built-in/Inport', [gcb, '/fltCC1sc'], 'Position', pos, 'Orientation', orient, 'OutDataTypeStr', 'single');
      | 
      |         pos = get_param(    [gcb, '/fltCC2sc'], 'Position');
      |         orient = get_param( [gcb, '/fltCC2sc'], 'Orientation');
      |         delete_block(       [gcb, '/fltCC2sc']);
      |         add_block('built-in/Inport', [gcb, '/fltCC2sc'], 'Position', pos, 'Orientation', orient, 'OutDataTypeStr', 'single');
      | 
      |         pos = get_param(    [gcb, '/fltAcc'], 'Position');
      |         orient = get_param( [gcb, '/fltAcc'], 'Orientation');
      |         delete_block(       [gcb, '/fltAcc']);
      |         add_block('built-in/Inport', [gcb, '/fltAcc'], 'Position', pos, 'Orientation', orient, 'OutDataTypeStr', 'single');
      | 
      |         pos = get_param(    [gcb, '/fltInErrK1'], 'Position');
      |         orient = get_param( [gcb, '/fltInErrK1'], 'Orientation');
      |         delete_block(       [gcb, '/fltInErrK1']);
      |         add_block('built-in/Inport', [gcb, '/fltInErrK1'], 'Position', pos, 'Orientation', orient, 'OutDataTypeStr', 'single');
      | 
      | 
      |         pos = get_param(    [gcb '/fltAcc_Out'], 'Position');
      |         orient = get_param( [gcb '/fltAcc_Out'], 'Orientation');
      |         delete_block(       [gcb '/fltAcc_Out']);
      |         add_block('built-in/Outport', [gcb '/fltAcc_Out'], 'Position', pos, 'Orientation', orient);
      | 
      |         pos = get_param(    [gcb '/fltInErrK1_Out'], 'Position');
      |         orient = get_param( [gcb '/fltInErrK1_Out'], 'Orientation');
      |         delete_block(       [gcb '/fltInErrK1_Out']);
      |         add_block('built-in/Outport', [gcb '/fltInErrK1_Out'], 'Position', pos, 'Orientation', orient);
      | 
      | 
      |         set_param([gcb '/fltInErr'], 'Port', '1');
      |         set_param([gcb '/fltControllerPIrOut_preset'], 'Port', '2');
      |         set_param([gcb '/fltCC1sc'], 'Port', '3');
      |         set_param([gcb '/fltCC2sc'], 'Port', '4');
      |         set_param([gcb '/fltAcc'], 'Port', '5');
      |         set_param([gcb '/fltInErrK1'], 'Port', '6');
      | 
      |         set_param([gcb '/fltOut'], 'Port', '1');
      |         set_param([gcb '/fltAcc_Out'], 'Port', '2');
      |         set_param([gcb '/fltInErrK1_Out'], 'Port', '3');
      | 
      |         set_param(gcb,'MaskEnables',{'on','on','off','off'});
      | 
      |         if (posblk(4) - posblk(2)) < 175
      |           height = 175;
      |           set_param(gcb,'Position',[posblk(1), posblk(2), posblk(3), posblk(2)+height])
      |         end
      |     end
      | end
      settings: RTWSystemCode=Inline
      mask Help: web([fileparts(which('ammclib_bam_S32K14x.slx')) '/../doc/S32K14XMCLUG.pdf'], '-browser')
      mask TypeOptions showStates: Hide (faster execution) | Show (allows debugging; connect feedback loops manually)
      mask Callback showStates:
      | maskStr = get_param(gcb,'showStates');
      | if strcmp(maskStr,'Hide (faster execution)'),
      |     set_param(gcb,'MaskEnables',{'on','on','on','on'});
      | else
      |     set_param(gcb,'MaskEnables',{'on','on','off','off'});
      | end
      mask TypeOptions resetStatesEnable: Pre-set according to the first set of inputs after reset | Clear to zero
      mask Display:
      | color('black');
      | pos = get_param(gcb, 'Position');
      | width = pos(3) - pos(1);
      | height = pos(4) - pos(2);
      | tX=width/2;
      | tY=height - 25;
      | color('black');
      | text(tX,tY, 'GFLIB_ControllerPIr_FLT', 'horizontalAlignment', 'center');
      | if showStates == 2
      |   color('red');
      |   text(tX,tY - 20, ['debugging mode' char(13) char(10) '(limited performance)'], 'horizontalAlignment', 'center');
      | end
  GFLIB_Cos_FLT : Subsystem  TreatAsAtomicUnit=on  mask(GFLIB_Cos_FLT){}
      mask help: Cosine function in single precision floating-point implementation. Refer to the AMMCLIB User's Guide for further details.
      mask init: same as ammclib_bam_S32K14x/GDFLIB/F16/GDFLIB_FilterFIR_F16
      settings: RTWSystemCode=Inline
      mask Help: web([fileparts(which('ammclib_bam_S32K14x.slx')) '/../doc/S32K14XMCLUG.pdf'], '-browser')
      mask Display: pos = get_param(gcb, 'Position');width = pos(3) - pos(1); height = pos(4) - pos(2);tX=width/2;tY=height - 8;color('black');text(tX,tY, 'GFLIB_Cos_FLT', 'horizontalAlignment', 'center');
  GFLIB_Hyst_FLT : Subsystem  TreatAsAtomicUnit=on  mask(GFLIB_Hyst_FLT){showStates=Hide (faster execution), fltHystOn=0, fltHystOff=0, fltOutValOn=0, fltOutValOff=0}
      mask prompts: showStates "Show internal states"; fltHystOn "fltHystOn (Value determining the upper threshold)"; fltHystOff "fltHystOff (Value determining the lower threshold)"; fltOutValOn "fltOutValOn (Value of the output when input is higher than the upper threshold)"; fltOutValOff "fltOutValOff (Value of the output when input is lower than the lower threshold)"
      mask help: Hysteresis function in single precision floating-point implementation. Refer to the AMMCLIB User's Guide for further details.
      mask init:
      | if ~evalin('base','exist(''tS8'',''var'')')
      |   if (2 ~= exist('SWLIBS_Typedefs.mat','file'))
      |       error('File SWLIBS_Typedefs.mat is not on the Matlab path. Please add the AMMCLIB "bam" folder in the Matlab Search Path.');
      |   else
      |       evalin('base', 'load(''SWLIBS_Typedefs.mat'')');
      |   end
      | end
      | if showStates == 1
      |     % hidden state variables
      |     if strcmp(get_param([gcb '/fltHystOn'], 'BlockType'), 'Inport')
      |         posblk = get_param(gcb, 'Position');
      | 
      |         pos = get_param(    [gcb, '/fltHystOn'], 'Position');
      |         orient = get_param( [gcb, '/fltHystOn'], 'Orientation');
      |         delete_block(       [gcb, '/fltHystOn']);
      |         add_block('built-in/Ground', [gcb, '/fltHystOn'], 'Position', pos, 'Orientation', orient);
      | 
      |         pos = get_param(    [gcb, '/fltHystOff'], 'Position');
      |         orient = get_param( [gcb, '/fltHystOff'], 'Orientation');
      |         delete_block(       [gcb, '/fltHystOff']);
      |         add_block('built-in/Ground', [gcb, '/fltHystOff'], 'Position', pos, 'Orientation', orient);
      | 
      |         pos = get_param(    [gcb, '/fltOutValOn'], 'Position');
      |         orient = get_param( [gcb, '/fltOutValOn'], 'Orientation');
      |         delete_block(       [gcb, '/fltOutValOn']);
      |         add_block('built-in/Ground', [gcb, '/fltOutValOn'], 'Position', pos, 'Orientation', orient);
      | 
      |         pos = get_param(    [gcb, '/fltOutValOff'], 'Position');
      |         orient = get_param( [gcb, '/fltOutValOff'], 'Orientation');
      |         delete_block(       [gcb, '/fltOutValOff']);
      |         add_block('built-in/Ground', [gcb, '/fltOutValOff'], 'Position', pos, 'Orientation', orient);
      | 
      |         pos = get_param(    [gcb, '/fltOutState'], 'Position');
      |         orient = get_param( [gcb, '/fltOutState'], 'Orientation');
      |         delete_block(       [gcb, '/fltOutState']);
      |         add_block('built-in/Ground', [gcb, '/fltOutState'], 'Position', pos, 'Orientation', orient);
      | 
      | 
      |         pos = get_param(    [gcb '/fltOutState_Out'], 'Position');
      |         orient = get_param( [gcb '/fltOutState_Out'], 'Orientation');
      |         delete_block(       [gcb '/fltOutState_Out']);
      |         add_block('built-in/Terminator', [gcb '/fltOutState_Out'], 'Position', pos, 'Orientation', orient);
      | 
      | 
      |         set_param([gcb '/fltIn'], 'Port', '1');
      | 
      |         set_param([gcb '/fltOut'], 'Port', '1');
      | 
      |         set_param(gcb,'MaskEnables',{'on','on','on','on','on'});
      | 
      |         if (posblk(4) - posblk(2)) > 50
      |           height = 50;
      |           set_param(gcb,'Position',[posblk(1), posblk(2), posblk(3), posblk(2)+height])
      |         end
      |     end
      | else
      |     % shown state variables
      |     if strcmp(get_param([gcb '/fltHystOn'], 'BlockType'), 'Ground')
      |         posblk = get_param(gcb, 'Position');
      | 
      |         pos = get_param(    [gcb, '/fltHystOn'], 'Position');
      |         orient = get_param( [gcb, '/fltHystOn'], 'Orientation');
      |         delete_block(       [gcb, '/fltHystOn']);
      |         add_block('built-in/Inport', [gcb, '/fltHystOn'], 'Position', pos, 'Orientation', orient, 'OutDataTypeStr', 'single');
      | 
      |         pos = get_param(    [gcb, '/fltHystOff'], 'Position');
      |         orient = get_param( [gcb, '/fltHystOff'], 'Orientation');
      |         delete_block(       [gcb, '/fltHystOff']);
      |         add_block('built-in/Inport', [gcb, '/fltHystOff'], 'Position', pos, 'Orientation', orient, 'OutDataTypeStr', 'single');
      | 
      |         pos = get_param(    [gcb, '/fltOutValOn'], 'Position');
      |         orient = get_param( [gcb, '/fltOutValOn'], 'Orientation');
      |         delete_block(       [gcb, '/fltOutValOn']);
      |         add_block('built-in/Inport', [gcb, '/fltOutValOn'], 'Position', pos, 'Orientation', orient, 'OutDataTypeStr', 'single');
      | 
      |         pos = get_param(    [gcb, '/fltOutValOff'], 'Position');
      |         orient = get_param( [gcb, '/fltOutValOff'], 'Orientation');
      |         delete_block(       [gcb, '/fltOutValOff']);
      |         add_block('built-in/Inport', [gcb, '/fltOutValOff'], 'Position', pos, 'Orientation', orient, 'OutDataTypeStr', 'single');
      | 
      |         pos = get_param(    [gcb, '/fltOutState'], 'Position');
      |         orient = get_param( [gcb, '/fltOutState'], 'Orientation');
      |         delete_block(       [gcb, '/fltOutState']);
      |         add_block('built-in/Inport', [gcb, '/fltOutState'], 'Position', pos, 'Orientation', orient, 'OutDataTypeStr', 'single');
      | 
      | 
      |         pos = get_param(    [gcb '/fltOutState_Out'], 'Position');
      |         orient = get_param( [gcb '/fltOutState_Out'], 'Orientation');
      |         delete_block(       [gcb '/fltOutState_Out']);
      |         add_block('built-in/Outport', [gcb '/fltOutState_Out'], 'Position', pos, 'Orientation', orient);
      | 
      | 
      |         set_param([gcb '/fltIn'], 'Port', '1');
      |         set_param([gcb '/fltHystOn'], 'Port', '2');
      |         set_param([gcb '/fltHystOff'], 'Port', '3');
      |         set_param([gcb '/fltOutValOn'], 'Port', '4');
      |         set_param([gcb '/fltOutValOff'], 'Port', '5');
      |         set_param([gcb '/fltOutState'], 'Port', '6');
      | 
      |         set_param([gcb '/fltOut'], 'Port', '1');
      |         set_param([gcb '/fltOutState_Out'], 'Port', '2');
      | 
      |         set_param(gcb,'MaskEnables',{'on','off','off','off','off'});
      | 
      |         if (posblk(4) - posblk(2)) < 175
      |           height = 175;
      |           set_param(gcb,'Position',[posblk(1), posblk(2), posblk(3), posblk(2)+height])
      |         end
      |     end
      | end
      settings: RTWSystemCode=Inline
      mask Help: web([fileparts(which('ammclib_bam_S32K14x.slx')) '/../doc/S32K14XMCLUG.pdf'], '-browser')
      mask TypeOptions showStates: Hide (faster execution) | Show (allows debugging; connect feedback loops manually)
      mask Callback showStates:
      | maskStr = get_param(gcb,'showStates');
      | if strcmp(maskStr,'Hide (faster execution)'),
      |     set_param(gcb,'MaskEnables',{'on','on','on','on','on'});
      | else
      |     set_param(gcb,'MaskEnables',{'on','off','off','off','off'});
      | end
      mask Display:
      | color('black');
      | pos = get_param(gcb, 'Position');
      | width = pos(3) - pos(1);
      | height = pos(4) - pos(2);
      | tX=width/2;
      | tY=height - 8;
      | color('black');
      | text(tX,tY, 'GFLIB_Hyst_FLT', 'horizontalAlignment', 'center');
      | if showStates == 2
      |   color('red');
      |   text(tX,tY - 20, ['debugging mode' char(13) char(10) '(limited performance)'], 'horizontalAlignment', 'center');
      | end
  GFLIB_IntegratorTR_FLT : Subsystem  TreatAsAtomicUnit=on  mask(GFLIB_IntegratorTR_FLT){showStates=Hide (faster execution), resetStatesEnable=Pre-set according to the first set of inputs after reset, fltC1=0}
      mask prompts: showStates "Show internal states"; resetStatesEnable "Internal state after reset"; fltC1 "fltC1 (Integrator coefficient)"
      mask help: Discrete integrator transformed from a linear model using Billinear (trapezoidal) transformation in single precision floating-point implementation. This block supports re-initialization of the internal state during simulation. If the block is reset, the integrator's output will be aligned with the input fltIntegratorTROut_preset. Refer to the AMMCLIB User's Guide for further details.
      mask init:
      | if ~evalin('base','exist(''tS8'',''var'')')
      |   if (2 ~= exist('SWLIBS_Typedefs.mat','file'))
      |       error('File SWLIBS_Typedefs.mat is not on the Matlab path. Please add the AMMCLIB "bam" folder in the Matlab Search Path.');
      |   else
      |       evalin('base', 'load(''SWLIBS_Typedefs.mat'')');
      |   end
      | end
      | if showStates == 1
      |     % hidden state variables
      |     if strcmp(get_param([gcb '/fltC1'], 'BlockType'), 'Inport')
      |         posblk = get_param(gcb, 'Position');
      | 
      |         pos = get_param(    [gcb, '/fltC1'], 'Position');
      |         orient = get_param( [gcb, '/fltC1'], 'Orientation');
      |         delete_block(       [gcb, '/fltC1']);
      |         add_block('built-in/Ground', [gcb, '/fltC1'], 'Position', pos, 'Orientation', orient);
      | 
      |         pos = get_param(    [gcb, '/fltState'], 'Position');
      |         orient = get_param( [gcb, '/fltState'], 'Orientation');
      |         delete_block(       [gcb, '/fltState']);
      |         add_block('built-in/Ground', [gcb, '/fltState'], 'Position', pos, 'Orientation', orient);
      | 
      |         pos = get_param(    [gcb, '/fltInK1'], 'Position');
      |         orient = get_param( [gcb, '/fltInK1'], 'Orientation');
      |         delete_block(       [gcb, '/fltInK1']);
      |         add_block('built-in/Ground', [gcb, '/fltInK1'], 'Position', pos, 'Orientation', orient);
      | 
      | 
      |         pos = get_param(    [gcb '/fltState_Out'], 'Position');
      |         orient = get_param( [gcb '/fltState_Out'], 'Orientation');
      |         delete_block(       [gcb '/fltState_Out']);
      |         add_block('built-in/Terminator', [gcb '/fltState_Out'], 'Position', pos, 'Orientation', orient);
      | 
      |         pos = get_param(    [gcb '/fltInK1_Out'], 'Position');
      |         orient = get_param( [gcb '/fltInK1_Out'], 'Orientation');
      |         delete_block(       [gcb '/fltInK1_Out']);
      |         add_block('built-in/Terminator', [gcb '/fltInK1_Out'], 'Position', pos, 'Orientation', orient);
      | 
      | 
      |         set_param([gcb '/fltIn'], 'Port', '1');
      |         set_param([gcb '/fltIntegratorTROut_preset'], 'Port', '2');
      | 
      |         set_param([gcb '/fltOut'], 'Port', '1');
      | 
      |         set_param(gcb,'MaskEnables',{'on','on','on'});
      | 
      |         if (posblk(4) - posblk(2)) > 75
      |           height = 75;
      |           set_param(gcb,'Position',[posblk(1), posblk(2), posblk(3), posblk(2)+height])
      |         end
      |     end
      | else
      |     % shown state variables
      |     if strcmp(get_param([gcb '/fltC1'], 'BlockType'), 'Ground')
      |         posblk = get_param(gcb, 'Position');
      | 
      |         pos = get_param(    [gcb, '/fltC1'], 'Position');
      |         orient = get_param( [gcb, '/fltC1'], 'Orientation');
      |         delete_block(       [gcb, '/fltC1']);
      |         add_block('built-in/Inport', [gcb, '/fltC1'], 'Position', pos, 'Orientation', orient, 'OutDataTypeStr', 'single');
      | 
      |         pos = get_param(    [gcb, '/fltState'], 'Position');
      |         orient = get_param( [gcb, '/fltState'], 'Orientation');
      |         delete_block(       [gcb, '/fltState']);
      |         add_block('built-in/Inport', [gcb, '/fltState'], 'Position', pos, 'Orientation', orient, 'OutDataTypeStr', 'single');
      | 
      |         pos = get_param(    [gcb, '/fltInK1'], 'Position');
      |         orient = get_param( [gcb, '/fltInK1'], 'Orientation');
      |         delete_block(       [gcb, '/fltInK1']);
      |         add_block('built-in/Inport', [gcb, '/fltInK1'], 'Position', pos, 'Orientation', orient, 'OutDataTypeStr', 'single');
      | 
      | 
      |         pos = get_param(    [gcb '/fltState_Out'], 'Position');
      |         orient = get_param( [gcb '/fltState_Out'], 'Orientation');
      |         delete_block(       [gcb '/fltState_Out']);
      |         add_block('built-in/Outport', [gcb '/fltState_Out'], 'Position', pos, 'Orientation', orient);
      | 
      |         pos = get_param(    [gcb '/fltInK1_Out'], 'Position');
      |         orient = get_param( [gcb '/fltInK1_Out'], 'Orientation');
      |         delete_block(       [gcb '/fltInK1_Out']);
      |         add_block('built-in/Outport', [gcb '/fltInK1_Out'], 'Position', pos, 'Orientation', orient);
      | 
      | 
      |         set_param([gcb '/fltIn'], 'Port', '1');
      |         set_param([gcb '/fltIntegratorTROut_preset'], 'Port', '2');
      |         set_param([gcb '/fltC1'], 'Port', '3');
      |         set_param([gcb '/fltState'], 'Port', '4');
      |         set_param([gcb '/fltInK1'], 'Port', '5');
      | 
      |         set_param([gcb '/fltOut'], 'Port', '1');
      |         set_param([gcb '/fltState_Out'], 'Port', '2');
      |         set_param([gcb '/fltInK1_Out'], 'Port', '3');
      | 
      |         set_param(gcb,'MaskEnables',{'on','on','off'});
      | 
      |         if (posblk(4) - posblk(2)) < 150
      |           height = 150;
      |           set_param(gcb,'Position',[posblk(1), posblk(2), posblk(3), posblk(2)+height])
      |         end
      |     end
      | end
      settings: RTWSystemCode=Inline
      mask Help: web([fileparts(which('ammclib_bam_S32K14x.slx')) '/../doc/S32K14XMCLUG.pdf'], '-browser')
      mask TypeOptions showStates: Hide (faster execution) | Show (allows debugging; connect feedback loops manually)
      mask Callback showStates:
      | maskStr = get_param(gcb,'showStates');
      | if strcmp(maskStr,'Hide (faster execution)'),
      |     set_param(gcb,'MaskEnables',{'on','on','on'});
      | else
      |     set_param(gcb,'MaskEnables',{'on','on','off'});
      | end
      mask TypeOptions resetStatesEnable: Pre-set according to the first set of inputs after reset | Clear to zero
      mask Display:
      | color('black');
      | pos = get_param(gcb, 'Position');
      | width = pos(3) - pos(1);
      | height = pos(4) - pos(2);
      | tX=width/2;
      | tY=height - 25;
      | color('black');
      | text(tX,tY, 'GFLIB_IntegratorTR_FLT', 'horizontalAlignment', 'center');
      | if showStates == 2
      |   color('red');
      |   text(tX,tY - 20, ['debugging mode' char(13) char(10) '(limited performance)'], 'horizontalAlignment', 'center');
      | end
  GFLIB_Limit_FLT : Subsystem  TreatAsAtomicUnit=on  mask(GFLIB_Limit_FLT){showStates=Hide (faster execution), fltLowerLimit=0, fltUpperLimit=0}
      mask prompts: showStates "Show internal states"; fltLowerLimit "fltLowerLimit (Lower limit)"; fltUpperLimit "fltUpperLimit (Upper limit)"
      mask help: Limit function in single precision floating-point implementation. Refer to the AMMCLIB User's Guide for further details.
      mask init:
      | if ~evalin('base','exist(''tS8'',''var'')')
      |   if (2 ~= exist('SWLIBS_Typedefs.mat','file'))
      |       error('File SWLIBS_Typedefs.mat is not on the Matlab path. Please add the AMMCLIB "bam" folder in the Matlab Search Path.');
      |   else
      |       evalin('base', 'load(''SWLIBS_Typedefs.mat'')');
      |   end
      | end
      | if showStates == 1
      |     % hidden state variables
      |     if strcmp(get_param([gcb '/fltLowerLimit'], 'BlockType'), 'Inport')
      |         posblk = get_param(gcb, 'Position');
      | 
      |         pos = get_param(    [gcb, '/fltLowerLimit'], 'Position');
      |         orient = get_param( [gcb, '/fltLowerLimit'], 'Orientation');
      |         delete_block(       [gcb, '/fltLowerLimit']);
      |         add_block('built-in/Ground', [gcb, '/fltLowerLimit'], 'Position', pos, 'Orientation', orient);
      | 
      |         pos = get_param(    [gcb, '/fltUpperLimit'], 'Position');
      |         orient = get_param( [gcb, '/fltUpperLimit'], 'Orientation');
      |         delete_block(       [gcb, '/fltUpperLimit']);
      |         add_block('built-in/Ground', [gcb, '/fltUpperLimit'], 'Position', pos, 'Orientation', orient);
      | 
      | 
      | 
      |         set_param([gcb '/fltIn'], 'Port', '1');
      | 
      |         set_param([gcb '/fltOut'], 'Port', '1');
      | 
      |         set_param(gcb,'MaskEnables',{'on','on','on'});
      | 
      |         if (posblk(4) - posblk(2)) > 50
      |           height = 50;
      |           set_param(gcb,'Position',[posblk(1), posblk(2), posblk(3), posblk(2)+height])
      |         end
      |     end
      | else
      |     % shown state variables
      |     if strcmp(get_param([gcb '/fltLowerLimit'], 'BlockType'), 'Ground')
      |         posblk = get_param(gcb, 'Position');
      | 
      |         pos = get_param(    [gcb, '/fltLowerLimit'], 'Position');
      |         orient = get_param( [gcb, '/fltLowerLimit'], 'Orientation');
      |         delete_block(       [gcb, '/fltLowerLimit']);
      |         add_block('built-in/Inport', [gcb, '/fltLowerLimit'], 'Position', pos, 'Orientation', orient, 'OutDataTypeStr', 'single');
      | 
      |         pos = get_param(    [gcb, '/fltUpperLimit'], 'Position');
      |         orient = get_param( [gcb, '/fltUpperLimit'], 'Orientation');
      |         delete_block(       [gcb, '/fltUpperLimit']);
      |         add_block('built-in/Inport', [gcb, '/fltUpperLimit'], 'Position', pos, 'Orientation', orient, 'OutDataTypeStr', 'single');
      | 
      | 
      | 
      |         set_param([gcb '/fltIn'], 'Port', '1');
      |         set_param([gcb '/fltLowerLimit'], 'Port', '2');
      |         set_param([gcb '/fltUpperLimit'], 'Port', '3');
      | 
      |         set_param([gcb '/fltOut'], 'Port', '1');
      | 
      |         set_param(gcb,'MaskEnables',{'on','off','off'});
      | 
      |         if (posblk(4) - posblk(2)) < 100
      |           height = 100;
      |           set_param(gcb,'Position',[posblk(1), posblk(2), posblk(3), posblk(2)+height])
      |         end
      |     end
      | end
      settings: RTWSystemCode=Inline
      mask Help: web([fileparts(which('ammclib_bam_S32K14x.slx')) '/../doc/S32K14XMCLUG.pdf'], '-browser')
      mask TypeOptions showStates: Hide (faster execution) | Show (allows debugging; connect feedback loops manually)
      mask Callback showStates:
      | maskStr = get_param(gcb,'showStates');
      | if strcmp(maskStr,'Hide (faster execution)'),
      |     set_param(gcb,'MaskEnables',{'on','on','on'});
      | else
      |     set_param(gcb,'MaskEnables',{'on','off','off'});
      | end
      mask Display:
      | color('black');
      | pos = get_param(gcb, 'Position');
      | width = pos(3) - pos(1);
      | height = pos(4) - pos(2);
      | tX=width/2;
      | tY=height - 8;
      | color('black');
      | text(tX,tY, 'GFLIB_Limit_FLT', 'horizontalAlignment', 'center');
      | if showStates == 2
      |   color('red');
      |   text(tX,tY - 20, ['debugging mode' char(13) char(10) '(limited performance)'], 'horizontalAlignment', 'center');
      | end
  GFLIB_Log10_FLT : Subsystem  TreatAsAtomicUnit=on  mask(GFLIB_Log10_FLT){}
      mask help: Fast base-10 logarithm function in single precision floating-point implementation. Refer to the AMMCLIB User's Guide for further details.
      mask init: same as ammclib_bam_S32K14x/GDFLIB/F16/GDFLIB_FilterFIR_F16
      settings: RTWSystemCode=Inline
      mask Help: web([fileparts(which('ammclib_bam_S32K14x.slx')) '/../doc/S32K14XMCLUG.pdf'], '-browser')
      mask Display: pos = get_param(gcb, 'Position');width = pos(3) - pos(1); height = pos(4) - pos(2);tX=width/2;tY=height - 8;color('black');text(tX,tY, 'GFLIB_Log10_FLT', 'horizontalAlignment', 'center');
  GFLIB_LowerLimit_FLT : Subsystem  TreatAsAtomicUnit=on  mask(GFLIB_LowerLimit_FLT){showStates=Hide (faster execution), fltLowerLimit=0}
      mask prompts: showStates "Show internal states"; fltLowerLimit "fltLowerLimit (Value determining the lower limit threshold)"
      mask help: Lower limit function in single precision floating-point implementation. Refer to the AMMCLIB User's Guide for further details.
      mask init:
      | if ~evalin('base','exist(''tS8'',''var'')')
      |   if (2 ~= exist('SWLIBS_Typedefs.mat','file'))
      |       error('File SWLIBS_Typedefs.mat is not on the Matlab path. Please add the AMMCLIB "bam" folder in the Matlab Search Path.');
      |   else
      |       evalin('base', 'load(''SWLIBS_Typedefs.mat'')');
      |   end
      | end
      | if showStates == 1
      |     % hidden state variables
      |     if strcmp(get_param([gcb '/fltLowerLimit'], 'BlockType'), 'Inport')
      |         posblk = get_param(gcb, 'Position');
      | 
      |         pos = get_param(    [gcb, '/fltLowerLimit'], 'Position');
      |         orient = get_param( [gcb, '/fltLowerLimit'], 'Orientation');
      |         delete_block(       [gcb, '/fltLowerLimit']);
      |         add_block('built-in/Ground', [gcb, '/fltLowerLimit'], 'Position', pos, 'Orientation', orient);
      | 
      | 
      | 
      |         set_param([gcb '/fltIn'], 'Port', '1');
      | 
      |         set_param([gcb '/fltOut'], 'Port', '1');
      | 
      |         set_param(gcb,'MaskEnables',{'on','on'});
      | 
      |         if (posblk(4) - posblk(2)) > 50
      |           height = 50;
      |           set_param(gcb,'Position',[posblk(1), posblk(2), posblk(3), posblk(2)+height])
      |         end
      |     end
      | else
      |     % shown state variables
      |     if strcmp(get_param([gcb '/fltLowerLimit'], 'BlockType'), 'Ground')
      |         posblk = get_param(gcb, 'Position');
      | 
      |         pos = get_param(    [gcb, '/fltLowerLimit'], 'Position');
      |         orient = get_param( [gcb, '/fltLowerLimit'], 'Orientation');
      |         delete_block(       [gcb, '/fltLowerLimit']);
      |         add_block('built-in/Inport', [gcb, '/fltLowerLimit'], 'Position', pos, 'Orientation', orient, 'OutDataTypeStr', 'single');
      | 
      | 
      | 
      |         set_param([gcb '/fltIn'], 'Port', '1');
      |         set_param([gcb '/fltLowerLimit'], 'Port', '2');
      | 
      |         set_param([gcb '/fltOut'], 'Port', '1');
      | 
      |         set_param(gcb,'MaskEnables',{'on','off'});
      | 
      |         if (posblk(4) - posblk(2)) < 75
      |           height = 75;
      |           set_param(gcb,'Position',[posblk(1), posblk(2), posblk(3), posblk(2)+height])
      |         end
      |     end
      | end
      settings: RTWSystemCode=Inline
      mask Help: web([fileparts(which('ammclib_bam_S32K14x.slx')) '/../doc/S32K14XMCLUG.pdf'], '-browser')
      mask TypeOptions showStates: Hide (faster execution) | Show (allows debugging; connect feedback loops manually)
      mask Callback showStates:
      | maskStr = get_param(gcb,'showStates');
      | if strcmp(maskStr,'Hide (faster execution)'),
      |     set_param(gcb,'MaskEnables',{'on','on'});
      | else
      |     set_param(gcb,'MaskEnables',{'on','off'});
      | end
      mask Display:
      | color('black');
      | pos = get_param(gcb, 'Position');
      | width = pos(3) - pos(1);
      | height = pos(4) - pos(2);
      | tX=width/2;
      | tY=height - 8;
      | color('black');
      | text(tX,tY, 'GFLIB_LowerLimit_FLT', 'horizontalAlignment', 'center');
      | if showStates == 2
      |   color('red');
      |   text(tX,tY - 20, ['debugging mode' char(13) char(10) '(limited performance)'], 'horizontalAlignment', 'center');
      | end
  GFLIB_Lut1D_FLT : Subsystem  TreatAsAtomicUnit=on  mask(GFLIB_Lut1D_FLT){pfltTable=[-0.75 -0.25 0.0 0.25 0.75], s32MidIdx=2}
      mask prompts: pfltTable "pfltTable (Vector holding the ordinate values of interpolating intervals)"; s32MidIdx "Middle index in the table pfltTable (zero-based indexing)"
      mask help: One dimensional lookup table function in single precision floating-point implementation. Refer to the AMMCLIB User's Guide for further details.
      mask init: same as ammclib_bam_S32K14x/GDFLIB/F16/GDFLIB_FilterFIR_F16
      settings: RTWSystemCode=Inline
      mask Help: web([fileparts(which('ammclib_bam_S32K14x.slx')) '/../doc/S32K14XMCLUG.pdf'], '-browser')
      mask Display: pos = get_param(gcb, 'Position');width = pos(3) - pos(1); height = pos(4) - pos(2);tX=width/2;tY=height - 8;color('black');text(tX,tY, 'GFLIB_Lut1D_FLT', 'horizontalAlignment', 'center');
  GFLIB_Lut2D_FLT : Subsystem  TreatAsAtomicUnit=on  mask(GFLIB_Lut2D_FLT){pfltTable=[-0.75 0.0 0.75; -0.5 0.0 0.5; -0.25 0.0 0.25], s32MidIdx=4}
      mask prompts: pfltTable "pfltTable (Matrix of z-coordinate values at vertices)"; s32MidIdx "Middle index in the table pfltTable (zero-based indexing over all elements)"
      mask help: Two dimensional lookup table function in single precision floating-point implementation. Refer to the AMMCLIB User's Guide for further details.
      mask init: same as ammclib_bam_S32K14x/GDFLIB/F16/GDFLIB_FilterFIR_F16
      settings: RTWSystemCode=Inline
      mask Help: web([fileparts(which('ammclib_bam_S32K14x.slx')) '/../doc/S32K14XMCLUG.pdf'], '-browser')
      mask Display: pos = get_param(gcb, 'Position');width = pos(3) - pos(1); height = pos(4) - pos(2);tX=width/2;tY=height - 8;color('black');text(tX,tY, 'GFLIB_Lut2D_FLT', 'horizontalAlignment', 'center');
  GFLIB_Ramp_FLT : Subsystem  TreatAsAtomicUnit=on  mask(GFLIB_Ramp_FLT){showStates=Hide (faster execution), fltRampUp=0, fltRampDown=0}
      mask prompts: showStates "Show internal states"; fltRampUp "fltRampUp (Ramp up increment coefficient)"; fltRampDown "fltRampDown (Ramp decrement coefficient)"
      mask help: Rate of change limiter - ramp function in single precision floating-point implementation. Refer to the AMMCLIB User's Guide for further details.
      mask init:
      | if ~evalin('base','exist(''tS8'',''var'')')
      |   if (2 ~= exist('SWLIBS_Typedefs.mat','file'))
      |       error('File SWLIBS_Typedefs.mat is not on the Matlab path. Please add the AMMCLIB "bam" folder in the Matlab Search Path.');
      |   else
      |       evalin('base', 'load(''SWLIBS_Typedefs.mat'')');
      |   end
      | end
      | if showStates == 1
      |     % hidden state variables
      |     if strcmp(get_param([gcb '/fltState'], 'BlockType'), 'Inport')
      |         posblk = get_param(gcb, 'Position');
      | 
      |         pos = get_param(    [gcb, '/fltState'], 'Position');
      |         orient = get_param( [gcb, '/fltState'], 'Orientation');
      |         delete_block(       [gcb, '/fltState']);
      |         add_block('built-in/Ground', [gcb, '/fltState'], 'Position', pos, 'Orientation', orient);
      | 
      |         pos = get_param(    [gcb, '/fltRampUp'], 'Position');
      |         orient = get_param( [gcb, '/fltRampUp'], 'Orientation');
      |         delete_block(       [gcb, '/fltRampUp']);
      |         add_block('built-in/Ground', [gcb, '/fltRampUp'], 'Position', pos, 'Orientation', orient);
      | 
      |         pos = get_param(    [gcb, '/fltRampDown'], 'Position');
      |         orient = get_param( [gcb, '/fltRampDown'], 'Orientation');
      |         delete_block(       [gcb, '/fltRampDown']);
      |         add_block('built-in/Ground', [gcb, '/fltRampDown'], 'Position', pos, 'Orientation', orient);
      | 
      | 
      |         pos = get_param(    [gcb '/fltState_Out'], 'Position');
      |         orient = get_param( [gcb '/fltState_Out'], 'Orientation');
      |         delete_block(       [gcb '/fltState_Out']);
      |         add_block('built-in/Terminator', [gcb '/fltState_Out'], 'Position', pos, 'Orientation', orient);
      | 
      | 
      |         set_param([gcb '/fltIn'], 'Port', '1');
      | 
      |         set_param([gcb '/fltOut'], 'Port', '1');
      | 
      |         set_param(gcb,'MaskEnables',{'on','on','on'});
      | 
      |         if (posblk(4) - posblk(2)) > 50
      |           height = 50;
      |           set_param(gcb,'Position',[posblk(1), posblk(2), posblk(3), posblk(2)+height])
      |         end
      |     end
      | else
      |     % shown state variables
      |     if strcmp(get_param([gcb '/fltState'], 'BlockType'), 'Ground')
      |         posblk = get_param(gcb, 'Position');
      | 
      |         pos = get_param(    [gcb, '/fltState'], 'Position');
      |         orient = get_param( [gcb, '/fltState'], 'Orientation');
      |         delete_block(       [gcb, '/fltState']);
      |         add_block('built-in/Inport', [gcb, '/fltState'], 'Position', pos, 'Orientation', orient, 'OutDataTypeStr', 'single');
      | 
      |         pos = get_param(    [gcb, '/fltRampUp'], 'Position');
      |         orient = get_param( [gcb, '/fltRampUp'], 'Orientation');
      |         delete_block(       [gcb, '/fltRampUp']);
      |         add_block('built-in/Inport', [gcb, '/fltRampUp'], 'Position', pos, 'Orientation', orient, 'OutDataTypeStr', 'single');
      | 
      |         pos = get_param(    [gcb, '/fltRampDown'], 'Position');
      |         orient = get_param( [gcb, '/fltRampDown'], 'Orientation');
      |         delete_block(       [gcb, '/fltRampDown']);
      |         add_block('built-in/Inport', [gcb, '/fltRampDown'], 'Position', pos, 'Orientation', orient, 'OutDataTypeStr', 'single');
      | 
      | 
      |         pos = get_param(    [gcb '/fltState_Out'], 'Position');
      |         orient = get_param( [gcb '/fltState_Out'], 'Orientation');
      |         delete_block(       [gcb '/fltState_Out']);
      |         add_block('built-in/Outport', [gcb '/fltState_Out'], 'Position', pos, 'Orientation', orient);
      | 
      | 
      |         set_param([gcb '/fltIn'], 'Port', '1');
      |         set_param([gcb '/fltState'], 'Port', '2');
      |         set_param([gcb '/fltRampUp'], 'Port', '3');
      |         set_param([gcb '/fltRampDown'], 'Port', '4');
      | 
      |         set_param([gcb '/fltOut'], 'Port', '1');
      |         set_param([gcb '/fltState_Out'], 'Port', '2');
      | 
      |         set_param(gcb,'MaskEnables',{'on','off','off'});
      | 
      |         if (posblk(4) - posblk(2)) < 125
      |           height = 125;
      |           set_param(gcb,'Position',[posblk(1), posblk(2), posblk(3), posblk(2)+height])
      |         end
      |     end
      | end
      settings: RTWSystemCode=Inline
      mask Help: web([fileparts(which('ammclib_bam_S32K14x.slx')) '/../doc/S32K14XMCLUG.pdf'], '-browser')
      mask TypeOptions showStates: Hide (faster execution) | Show (allows debugging; connect feedback loops manually)
      mask Callback showStates:
      | maskStr = get_param(gcb,'showStates');
      | if strcmp(maskStr,'Hide (faster execution)'),
      |     set_param(gcb,'MaskEnables',{'on','on','on'});
      | else
      |     set_param(gcb,'MaskEnables',{'on','off','off'});
      | end
      mask Display:
      | color('black');
      | pos = get_param(gcb, 'Position');
      | width = pos(3) - pos(1);
      | height = pos(4) - pos(2);
      | tX=width/2;
      | tY=height - 8;
      | color('black');
      | text(tX,tY, 'GFLIB_Ramp_FLT', 'horizontalAlignment', 'center');
      | if showStates == 2
      |   color('red');
      |   text(tX,tY - 20, ['debugging mode' char(13) char(10) '(limited performance)'], 'horizontalAlignment', 'center');
      | end
  GFLIB_Sign_FLT : Subsystem  TreatAsAtomicUnit=on  mask(GFLIB_Sign_FLT){}
      mask help: Sign function in single precision floating-point implementation. Refer to the AMMCLIB User's Guide for further details.
      mask init: same as ammclib_bam_S32K14x/GDFLIB/F16/GDFLIB_FilterFIR_F16
      settings: RTWSystemCode=Inline
      mask Help: web([fileparts(which('ammclib_bam_S32K14x.slx')) '/../doc/S32K14XMCLUG.pdf'], '-browser')
      mask Display: pos = get_param(gcb, 'Position');width = pos(3) - pos(1); height = pos(4) - pos(2);tX=width/2;tY=height - 8;color('black');text(tX,tY, 'GFLIB_Sign_FLT', 'horizontalAlignment', 'center');
  GFLIB_SinCos_FLT : Subsystem  TreatAsAtomicUnit=on  mask(GFLIB_SinCos_FLT){}
      mask help: Calculation of sine and cosine of the same argument in single precision floating-point implementation. Refer to the AMMCLIB User's Guide for further details.
      mask init: same as ammclib_bam_S32K14x/GDFLIB/F16/GDFLIB_FilterFIR_F16
      settings: RTWSystemCode=Inline
      mask Help: web([fileparts(which('ammclib_bam_S32K14x.slx')) '/../doc/S32K14XMCLUG.pdf'], '-browser')
      mask Display: pos = get_param(gcb, 'Position');width = pos(3) - pos(1); height = pos(4) - pos(2);tX=width/2;tY=height - 8;color('black');text(tX,tY, 'GFLIB_SinCos_FLT', 'horizontalAlignment', 'center');
  GFLIB_Sin_FLT : Subsystem  TreatAsAtomicUnit=on  mask(GFLIB_Sin_FLT){}
      mask help: Sine function in single precision floating-point implementation. Refer to the AMMCLIB User's Guide for further details.
      mask init: same as ammclib_bam_S32K14x/GDFLIB/F16/GDFLIB_FilterFIR_F16
      settings: RTWSystemCode=Inline
      mask Help: web([fileparts(which('ammclib_bam_S32K14x.slx')) '/../doc/S32K14XMCLUG.pdf'], '-browser')
      mask Display: pos = get_param(gcb, 'Position');width = pos(3) - pos(1); height = pos(4) - pos(2);tX=width/2;tY=height - 8;color('black');text(tX,tY, 'GFLIB_Sin_FLT', 'horizontalAlignment', 'center');
  GFLIB_Sqrt_FLT : Subsystem  TreatAsAtomicUnit=on  mask(GFLIB_Sqrt_FLT){}
      mask help: Square root approximation in single precision floating-point implementation. Refer to the AMMCLIB User's Guide for further details.
      mask init: same as ammclib_bam_S32K14x/GDFLIB/F16/GDFLIB_FilterFIR_F16
      settings: RTWSystemCode=Inline
      mask Help: web([fileparts(which('ammclib_bam_S32K14x.slx')) '/../doc/S32K14XMCLUG.pdf'], '-browser')
      mask Display: pos = get_param(gcb, 'Position');width = pos(3) - pos(1); height = pos(4) - pos(2);tX=width/2;tY=height - 8;color('black');text(tX,tY, 'GFLIB_Sqrt_FLT', 'horizontalAlignment', 'center');
  GFLIB_Tan_FLT : Subsystem  TreatAsAtomicUnit=on  mask(GFLIB_Tan_FLT){}
      mask help: Tangent function in single precision floating-point implementation. Refer to the AMMCLIB User's Guide for further details.
      mask init: same as ammclib_bam_S32K14x/GDFLIB/F16/GDFLIB_FilterFIR_F16
      settings: RTWSystemCode=Inline
      mask Help: web([fileparts(which('ammclib_bam_S32K14x.slx')) '/../doc/S32K14XMCLUG.pdf'], '-browser')
      mask Display: pos = get_param(gcb, 'Position');width = pos(3) - pos(1); height = pos(4) - pos(2);tX=width/2;tY=height - 8;color('black');text(tX,tY, 'GFLIB_Tan_FLT', 'horizontalAlignment', 'center');
  GFLIB_UpperLimit_FLT : Subsystem  TreatAsAtomicUnit=on  mask(GFLIB_UpperLimit_FLT){showStates=Hide (faster execution), fltUpperLimit=0}
      mask prompts: showStates "Show internal states"; fltUpperLimit "fltUpperLimit (Value determining the upper limit threshold)"
      mask help: Upper limit function in single precision floating-point implementation. Refer to the AMMCLIB User's Guide for further details.
      mask init:
      | if ~evalin('base','exist(''tS8'',''var'')')
      |   if (2 ~= exist('SWLIBS_Typedefs.mat','file'))
      |       error('File SWLIBS_Typedefs.mat is not on the Matlab path. Please add the AMMCLIB "bam" folder in the Matlab Search Path.');
      |   else
      |       evalin('base', 'load(''SWLIBS_Typedefs.mat'')');
      |   end
      | end
      | if showStates == 1
      |     % hidden state variables
      |     if strcmp(get_param([gcb '/fltUpperLimit'], 'BlockType'), 'Inport')
      |         posblk = get_param(gcb, 'Position');
      | 
      |         pos = get_param(    [gcb, '/fltUpperLimit'], 'Position');
      |         orient = get_param( [gcb, '/fltUpperLimit'], 'Orientation');
      |         delete_block(       [gcb, '/fltUpperLimit']);
      |         add_block('built-in/Ground', [gcb, '/fltUpperLimit'], 'Position', pos, 'Orientation', orient);
      | 
      | 
      | 
      |         set_param([gcb '/fltIn'], 'Port', '1');
      | 
      |         set_param([gcb '/fltOut'], 'Port', '1');
      | 
      |         set_param(gcb,'MaskEnables',{'on','on'});
      | 
      |         if (posblk(4) - posblk(2)) > 50
      |           height = 50;
      |           set_param(gcb,'Position',[posblk(1), posblk(2), posblk(3), posblk(2)+height])
      |         end
      |     end
      | else
      |     % shown state variables
      |     if strcmp(get_param([gcb '/fltUpperLimit'], 'BlockType'), 'Ground')
      |         posblk = get_param(gcb, 'Position');
      | 
      |         pos = get_param(    [gcb, '/fltUpperLimit'], 'Position');
      |         orient = get_param( [gcb, '/fltUpperLimit'], 'Orientation');
      |         delete_block(       [gcb, '/fltUpperLimit']);
      |         add_block('built-in/Inport', [gcb, '/fltUpperLimit'], 'Position', pos, 'Orientation', orient, 'OutDataTypeStr', 'single');
      | 
      | 
      | 
      |         set_param([gcb '/fltIn'], 'Port', '1');
      |         set_param([gcb '/fltUpperLimit'], 'Port', '2');
      | 
      |         set_param([gcb '/fltOut'], 'Port', '1');
      | 
      |         set_param(gcb,'MaskEnables',{'on','off'});
      | 
      |         if (posblk(4) - posblk(2)) < 75
      |           height = 75;
      |           set_param(gcb,'Position',[posblk(1), posblk(2), posblk(3), posblk(2)+height])
      |         end
      |     end
      | end
      settings: RTWSystemCode=Inline
      mask Help: web([fileparts(which('ammclib_bam_S32K14x.slx')) '/../doc/S32K14XMCLUG.pdf'], '-browser')
      mask TypeOptions showStates: Hide (faster execution) | Show (allows debugging; connect feedback loops manually)
      mask Callback showStates:
      | maskStr = get_param(gcb,'showStates');
      | if strcmp(maskStr,'Hide (faster execution)'),
      |     set_param(gcb,'MaskEnables',{'on','on'});
      | else
      |     set_param(gcb,'MaskEnables',{'on','off'});
      | end
      mask Display:
      | color('black');
      | pos = get_param(gcb, 'Position');
      | width = pos(3) - pos(1);
      | height = pos(4) - pos(2);
      | tX=width/2;
      | tY=height - 8;
      | color('black');
      | text(tX,tY, 'GFLIB_UpperLimit_FLT', 'horizontalAlignment', 'center');
      | if showStates == 2
      |   color('red');
      |   text(tX,tY - 20, ['debugging mode' char(13) char(10) '(limited performance)'], 'horizontalAlignment', 'center');
      | end
  GFLIB_VLog10_FLT : Subsystem  TreatAsAtomicUnit=on  mask(GFLIB_VLog10_FLT){}
      mask help: Single precision floating-point implementation of the GFLIB_VLog10 function, which computes base-10 logarithm of all elements of a vector. Refer to the AMMCLIB User's Guide for further details.
      mask init: same as ammclib_bam_S32K14x/GDFLIB/F16/GDFLIB_FilterFIR_F16
      settings: RTWSystemCode=Inline
      mask Help: web([fileparts(which('ammclib_bam_S32K14x.slx')) '/../doc/S32K14XMCLUG.pdf'], '-browser')
      mask Display: pos = get_param(gcb, 'Position');width = pos(3) - pos(1); height = pos(4) - pos(2);tX=width/2;tY=height - 8;color('black');text(tX,tY, 'GFLIB_VLog10_FLT', 'horizontalAlignment', 'center');
  GFLIB_VMin_FLT : Subsystem  TreatAsAtomicUnit=on  mask(GFLIB_VMin_FLT){}
      mask help: Single precision floating-point implementation of the GFLIB_VMin function, which finds the index of a vector minimum. Refer to the AMMCLIB User's Guide for further details.
      mask init: same as ammclib_bam_S32K14x/GDFLIB/F16/GDFLIB_FilterFIR_F16
      settings: RTWSystemCode=Inline
      mask Help: web([fileparts(which('ammclib_bam_S32K14x.slx')) '/../doc/S32K14XMCLUG.pdf'], '-browser')
      mask Display: pos = get_param(gcb, 'Position');width = pos(3) - pos(1); height = pos(4) - pos(2);tX=width/2;tY=height - 8;color('black');text(tX,tY, 'GFLIB_VMin_FLT', 'horizontalAlignment', 'center');
  GFLIB_VectorLimit_FLT : Subsystem  TreatAsAtomicUnit=on  mask(GFLIB_VectorLimit_FLT){showStates=Hide (faster execution), fltLimit=0}
      mask prompts: showStates "Show internal states"; fltLimit "fltLimit (The maximum magnitude of the input 2-element vector)"
      mask help: Single precision floating-point implementation of the GFLIB_VectorLimit function which limits the magnitude of the input 2-element vector, keeping its direction unchanged. Refer to the AMMCLIB User's Guide for further details.
      mask init:
      | if ~evalin('base','exist(''tS8'',''var'')')
      |   if (2 ~= exist('SWLIBS_Typedefs.mat','file'))
      |       error('File SWLIBS_Typedefs.mat is not on the Matlab path. Please add the AMMCLIB "bam" folder in the Matlab Search Path.');
      |   else
      |       evalin('base', 'load(''SWLIBS_Typedefs.mat'')');
      |   end
      | end
      | if showStates == 1
      |     % hidden state variables
      |     if strcmp(get_param([gcb '/fltLimit'], 'BlockType'), 'Inport')
      |         posblk = get_param(gcb, 'Position');
      | 
      |         pos = get_param(    [gcb, '/fltLimit'], 'Position');
      |         orient = get_param( [gcb, '/fltLimit'], 'Orientation');
      |         delete_block(       [gcb, '/fltLimit']);
      |         add_block('built-in/Ground', [gcb, '/fltLimit'], 'Position', pos, 'Orientation', orient);
      | 
      | 
      | 
      |         set_param([gcb '/pIn'], 'Port', '1');
      | 
      |         set_param([gcb '/bFlag'], 'Port', '1');
      |         set_param([gcb '/pOut'], 'Port', '2');
      | 
      |         set_param(gcb,'MaskEnables',{'on','on'});
      | 
      |         if (posblk(4) - posblk(2)) > 75
      |           height = 75;
      |           set_param(gcb,'Position',[posblk(1), posblk(2), posblk(3), posblk(2)+height])
      |         end
      |     end
      | else
      |     % shown state variables
      |     if strcmp(get_param([gcb '/fltLimit'], 'BlockType'), 'Ground')
      |         posblk = get_param(gcb, 'Position');
      | 
      |         pos = get_param(    [gcb, '/fltLimit'], 'Position');
      |         orient = get_param( [gcb, '/fltLimit'], 'Orientation');
      |         delete_block(       [gcb, '/fltLimit']);
      |         add_block('built-in/Inport', [gcb, '/fltLimit'], 'Position', pos, 'Orientation', orient, 'OutDataTypeStr', 'single');
      | 
      | 
      | 
      |         set_param([gcb '/pIn'], 'Port', '1');
      |         set_param([gcb '/fltLimit'], 'Port', '2');
      | 
      |         set_param([gcb '/bFlag'], 'Port', '1');
      |         set_param([gcb '/pOut'], 'Port', '2');
      | 
      |         set_param(gcb,'MaskEnables',{'on','off'});
      | 
      |         if (posblk(4) - posblk(2)) < 75
      |           height = 75;
      |           set_param(gcb,'Position',[posblk(1), posblk(2), posblk(3), posblk(2)+height])
      |         end
      |     end
      | end
      settings: RTWSystemCode=Inline
      mask Help: web([fileparts(which('ammclib_bam_S32K14x.slx')) '/../doc/S32K14XMCLUG.pdf'], '-browser')
      mask TypeOptions showStates: Hide (faster execution) | Show (allows debugging; connect feedback loops manually)
      mask Callback showStates:
      | maskStr = get_param(gcb,'showStates');
      | if strcmp(maskStr,'Hide (faster execution)'),
      |     set_param(gcb,'MaskEnables',{'on','on'});
      | else
      |     set_param(gcb,'MaskEnables',{'on','off'});
      | end
      mask Display:
      | color('black');
      | pos = get_param(gcb, 'Position');
      | width = pos(3) - pos(1);
      | height = pos(4) - pos(2);
      | tX=width/2;
      | tY=height - 8;
      | color('black');
      | text(tX,tY, 'GFLIB_VectorLimit_FLT', 'horizontalAlignment', 'center');
      | if showStates == 2
      |   color('red');
      |   text(tX,tY - 20, ['debugging mode' char(13) char(10) '(limited performance)'], 'horizontalAlignment', 'center');
      | end
